simulink model "OR_6s_30l"  (R2023b)
settings: Solver=VariableStepAuto  StartTime=0.0  StopTime=10.0  RelTol=1e-3
libraries: ABB_UPPAAL_Library x76
(part 1 of 2)
settings Model: Creator=francescopellei  LastModifiedBy=francescopellei

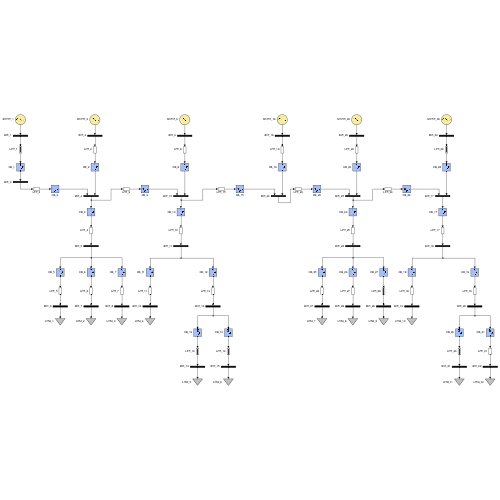
[thumbnail: Simulink's stored preview of the top-level diagram]
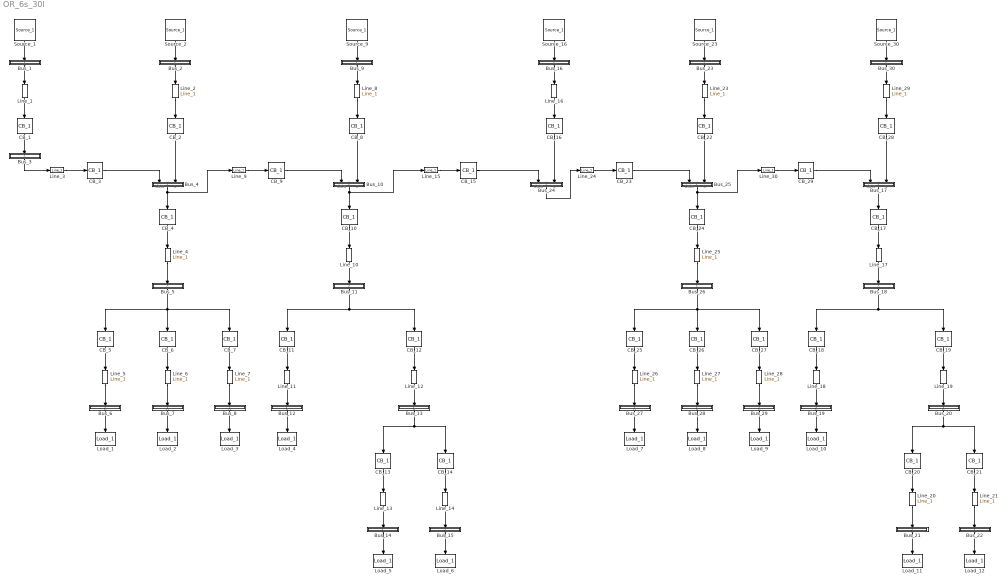
== system OR_6s_30l ==
  Bus_1 : MATLAB Function  TreatAsAtomicUnit=on  mask{MyInitialization=0, Bus_ID=1, Fault_flag=1}
      mask prompts: Bus_ID "Bus ID"; Fault_flag "Fault flag"
      settings: CopyFcn=|
      | Component_Name = get_param(gcb, 'Name');
      | set_param(gcb, 'Bus_ID', num2str(strtrim(extractAfter(Component_Name, '_'))));
      | 
      | blocks = find_system(gcs, 'SearchDepth', 1, 'Type', 'Block');
      | 
      | for k = 1:length(blocks)
      |     if contains(extractAfter(blocks{k,1}, '/'), 'Source')
      |         set_param(blocks{k}, 'BackgroundColor', '[0.929000, 0.490000, 0.439000]');
      |     end
      | end
      settings: NameChangeFcn=|
      | Component_Name = get_param(gcb, 'Name');
      | old_ID = get_param(gcb, 'Bus_ID');
      | 
      | pattern = '_\d+';
      | match = regexp(Component_Name, pattern, 'match');
      | 
      | if ~isempty(match)
      |     if ~isequal(old_ID, num2str(strtrim(extractAfter(Component_Name, '_'))))
      |         set_param(gcb, 'Bus_ID', num2str(strtrim(extractAfter(Component_Name, '_'))));
      |     end
      | else
      |     newName = [Component_Name '_' old_ID];
      |     set_param(gcb, 'Name', newName);
      | end
      | 
      | if ~isequal(old_ID, get_param(gcb, 'Bus_ID'))
      | 
      |     data = get_param(gcb, 'PortConnectivity');
      |     for i = 1:numel(data)
      |         sourceHandle = data(i,1).SrcBlock;
      |         if ~isempty(sourceHandle) && sourceHandle ~= -1
      |             sourceParams = get_param(sourceHandle, 'DialogParameters');
      |             fn = fieldnames(sourceParams);
      |             if contains(fn{2}, 'Source')
      |                 Bus_ID = get_param(gcb, 'Bus_ID');
      |                 set_param(sourceHandle, 'Source_ID', Bus_ID);
      |             end
      |         end
      |     end
      | 
      |     blocks = find_system(gcs, 'SearchDepth', 1, 'Type', 'Block');
      | 
      |     for k = 1:length(blocks)
      |         if contains(extractAfter(blocks{k,1}, '/'), 'Source')
      |             set_param(blocks{k}, 'BackgroundColor', '[0.929000, 0.490000, 0.439000]');
      |         end
      |     end
      | 
      | end
      settings: PreDeleteFcn=|
      | blocks = find_system(gcs, 'SearchDepth', 1, 'Type', 'Block');
      | 
      | for k = 1:length(blocks)
      |     if contains(extractAfter(blocks{k,1}, '/'), 'Source')
      |         set_param(blocks{k}, 'BackgroundColor', '[0.929000, 0.490000, 0.439000]');
      |     end
      | end
  Bus_10 : MATLAB Function  TreatAsAtomicUnit=on  mask{MyInitialization=0, Bus_ID=10, Fault_flag=1}
      mask prompts: Bus_ID "Bus ID"; Fault_flag "Fault flag"
      settings: CopyFcn=|
      | Component_Name = get_param(gcb, 'Name');
      | set_param(gcb, 'Bus_ID', num2str(strtrim(extractAfter(Component_Name, '_'))));
      | 
      | blocks = find_system(gcs, 'SearchDepth', 1, 'Type', 'Block');
      | 
      | for k = 1:length(blocks)
      |     if contains(extractAfter(blocks{k,1}, '/'), 'Source')
      |         set_param(blocks{k}, 'BackgroundColor', '[0.929000, 0.490000, 0.439000]');
      |     end
      | end
      settings: NameChangeFcn=|
      | Component_Name = get_param(gcb, 'Name');
      | old_ID = get_param(gcb, 'Bus_ID');
      | 
      | pattern = '_\d+';
      | match = regexp(Component_Name, pattern, 'match');
      | 
      | if ~isempty(match)
      |     if ~isequal(old_ID, num2str(strtrim(extractAfter(Component_Name, '_'))))
      |         set_param(gcb, 'Bus_ID', num2str(strtrim(extractAfter(Component_Name, '_'))));
      |     end
      | else
      |     newName = [Component_Name '_' old_ID];
      |     set_param(gcb, 'Name', newName);
      | end
      | 
      | if ~isequal(old_ID, get_param(gcb, 'Bus_ID'))
      | 
      |     data = get_param(gcb, 'PortConnectivity');
      |     for i = 1:numel(data)
      |         sourceHandle = data(i,1).SrcBlock;
      |         if ~isempty(sourceHandle) && sourceHandle ~= -1
      |             sourceParams = get_param(sourceHandle, 'DialogParameters');
      |             fn = fieldnames(sourceParams);
      |             if contains(fn{2}, 'Source')
      |                 Bus_ID = get_param(gcb, 'Bus_ID');
      |                 set_param(sourceHandle, 'Source_ID', Bus_ID);
      |             end
      |         end
      |     end
      | 
      |     blocks = find_system(gcs, 'SearchDepth', 1, 'Type', 'Block');
      | 
      |     for k = 1:length(blocks)
      |         if contains(extractAfter(blocks{k,1}, '/'), 'Source')
      |             set_param(blocks{k}, 'BackgroundColor', '[0.929000, 0.490000, 0.439000]');
      |         end
      |     end
      | 
      | end
      settings: PreDeleteFcn=|
      | blocks = find_system(gcs, 'SearchDepth', 1, 'Type', 'Block');
      | 
      | for k = 1:length(blocks)
      |     if contains(extractAfter(blocks{k,1}, '/'), 'Source')
      |         set_param(blocks{k}, 'BackgroundColor', '[0.929000, 0.490000, 0.439000]');
      |     end
      | end
  Bus_11 : MATLAB Function  TreatAsAtomicUnit=on  mask{MyInitialization=0, Bus_ID=11, Fault_flag=1}
      mask prompts: Bus_ID "Bus ID"; Fault_flag "Fault flag"
      settings: CopyFcn=|
      | Component_Name = get_param(gcb, 'Name');
      | set_param(gcb, 'Bus_ID', num2str(strtrim(extractAfter(Component_Name, '_'))));
      | 
      | blocks = find_system(gcs, 'SearchDepth', 1, 'Type', 'Block');
      | 
      | for k = 1:length(blocks)
      |     if contains(extractAfter(blocks{k,1}, '/'), 'Source')
      |         set_param(blocks{k}, 'BackgroundColor', '[0.929000, 0.490000, 0.439000]');
      |     end
      | end
      settings: NameChangeFcn=|
      | Component_Name = get_param(gcb, 'Name');
      | old_ID = get_param(gcb, 'Bus_ID');
      | 
      | pattern = '_\d+';
      | match = regexp(Component_Name, pattern, 'match');
      | 
      | if ~isempty(match)
      |     if ~isequal(old_ID, num2str(strtrim(extractAfter(Component_Name, '_'))))
      |         set_param(gcb, 'Bus_ID', num2str(strtrim(extractAfter(Component_Name, '_'))));
      |     end
      | else
      |     newName = [Component_Name '_' old_ID];
      |     set_param(gcb, 'Name', newName);
      | end
      | 
      | if ~isequal(old_ID, get_param(gcb, 'Bus_ID'))
      | 
      |     data = get_param(gcb, 'PortConnectivity');
      |     for i = 1:numel(data)
      |         sourceHandle = data(i,1).SrcBlock;
      |         if ~isempty(sourceHandle) && sourceHandle ~= -1
      |             sourceParams = get_param(sourceHandle, 'DialogParameters');
      |             fn = fieldnames(sourceParams);
      |             if contains(fn{2}, 'Source')
      |                 Bus_ID = get_param(gcb, 'Bus_ID');
      |                 set_param(sourceHandle, 'Source_ID', Bus_ID);
      |             end
      |         end
      |     end
      | 
      |     blocks = find_system(gcs, 'SearchDepth', 1, 'Type', 'Block');
      | 
      |     for k = 1:length(blocks)
      |         if contains(extractAfter(blocks{k,1}, '/'), 'Source')
      |             set_param(blocks{k}, 'BackgroundColor', '[0.929000, 0.490000, 0.439000]');
      |         end
      |     end
      | 
      | end
      settings: PreDeleteFcn=|
      | blocks = find_system(gcs, 'SearchDepth', 1, 'Type', 'Block');
      | 
      | for k = 1:length(blocks)
      |     if contains(extractAfter(blocks{k,1}, '/'), 'Source')
      |         set_param(blocks{k}, 'BackgroundColor', '[0.929000, 0.490000, 0.439000]');
      |     end
      | end
  Bus_12 : MATLAB Function  TreatAsAtomicUnit=on  mask{MyInitialization=0, Bus_ID=12, Fault_flag=1}
      mask prompts: Bus_ID "Bus ID"; Fault_flag "Fault flag"
      settings: CopyFcn=|
      | Component_Name = get_param(gcb, 'Name');
      | set_param(gcb, 'Bus_ID', num2str(strtrim(extractAfter(Component_Name, '_'))));
      | 
      | blocks = find_system(gcs, 'SearchDepth', 1, 'Type', 'Block');
      | 
      | for k = 1:length(blocks)
      |     if contains(extractAfter(blocks{k,1}, '/'), 'Source')
      |         set_param(blocks{k}, 'BackgroundColor', '[0.929000, 0.490000, 0.439000]');
      |     end
      | end
      settings: NameChangeFcn=|
      | Component_Name = get_param(gcb, 'Name');
      | old_ID = get_param(gcb, 'Bus_ID');
      | 
      | pattern = '_\d+';
      | match = regexp(Component_Name, pattern, 'match');
      | 
      | if ~isempty(match)
      |     if ~isequal(old_ID, num2str(strtrim(extractAfter(Component_Name, '_'))))
      |         set_param(gcb, 'Bus_ID', num2str(strtrim(extractAfter(Component_Name, '_'))));
      |     end
      | else
      |     newName = [Component_Name '_' old_ID];
      |     set_param(gcb, 'Name', newName);
      | end
      | 
      | if ~isequal(old_ID, get_param(gcb, 'Bus_ID'))
      | 
      |     data = get_param(gcb, 'PortConnectivity');
      |     for i = 1:numel(data)
      |         sourceHandle = data(i,1).SrcBlock;
      |         if ~isempty(sourceHandle) && sourceHandle ~= -1
      |             sourceParams = get_param(sourceHandle, 'DialogParameters');
      |             fn = fieldnames(sourceParams);
      |             if contains(fn{2}, 'Source')
      |                 Bus_ID = get_param(gcb, 'Bus_ID');
      |                 set_param(sourceHandle, 'Source_ID', Bus_ID);
      |             end
      |         end
      |     end
      | 
      |     blocks = find_system(gcs, 'SearchDepth', 1, 'Type', 'Block');
      | 
      |     for k = 1:length(blocks)
      |         if contains(extractAfter(blocks{k,1}, '/'), 'Source')
      |             set_param(blocks{k}, 'BackgroundColor', '[0.929000, 0.490000, 0.439000]');
      |         end
      |     end
      | 
      | end
      settings: PreDeleteFcn=|
      | blocks = find_system(gcs, 'SearchDepth', 1, 'Type', 'Block');
      | 
      | for k = 1:length(blocks)
      |     if contains(extractAfter(blocks{k,1}, '/'), 'Source')
      |         set_param(blocks{k}, 'BackgroundColor', '[0.929000, 0.490000, 0.439000]');
      |     end
      | end
  Bus_13 : MATLAB Function  TreatAsAtomicUnit=on  mask{MyInitialization=0, Bus_ID=13, Fault_flag=1}
      mask prompts: Bus_ID "Bus ID"; Fault_flag "Fault flag"
      settings: CopyFcn=|
      | Component_Name = get_param(gcb, 'Name');
      | set_param(gcb, 'Bus_ID', num2str(strtrim(extractAfter(Component_Name, '_'))));
      | 
      | blocks = find_system(gcs, 'SearchDepth', 1, 'Type', 'Block');
      | 
      | for k = 1:length(blocks)
      |     if contains(extractAfter(blocks{k,1}, '/'), 'Source')
      |         set_param(blocks{k}, 'BackgroundColor', '[0.929000, 0.490000, 0.439000]');
      |     end
      | end
      settings: NameChangeFcn=|
      | Component_Name = get_param(gcb, 'Name');
      | old_ID = get_param(gcb, 'Bus_ID');
      | 
      | pattern = '_\d+';
      | match = regexp(Component_Name, pattern, 'match');
      | 
      | if ~isempty(match)
      |     if ~isequal(old_ID, num2str(strtrim(extractAfter(Component_Name, '_'))))
      |         set_param(gcb, 'Bus_ID', num2str(strtrim(extractAfter(Component_Name, '_'))));
      |     end
      | else
      |     newName = [Component_Name '_' old_ID];
      |     set_param(gcb, 'Name', newName);
      | end
      | 
      | if ~isequal(old_ID, get_param(gcb, 'Bus_ID'))
      | 
      |     data = get_param(gcb, 'PortConnectivity');
      |     for i = 1:numel(data)
      |         sourceHandle = data(i,1).SrcBlock;
      |         if ~isempty(sourceHandle) && sourceHandle ~= -1
      |             sourceParams = get_param(sourceHandle, 'DialogParameters');
      |             fn = fieldnames(sourceParams);
      |             if contains(fn{2}, 'Source')
      |                 Bus_ID = get_param(gcb, 'Bus_ID');
      |                 set_param(sourceHandle, 'Source_ID', Bus_ID);
      |             end
      |         end
      |     end
      | 
      |     blocks = find_system(gcs, 'SearchDepth', 1, 'Type', 'Block');
      | 
      |     for k = 1:length(blocks)
      |         if contains(extractAfter(blocks{k,1}, '/'), 'Source')
      |             set_param(blocks{k}, 'BackgroundColor', '[0.929000, 0.490000, 0.439000]');
      |         end
      |     end
      | 
      | end
      settings: PreDeleteFcn=|
      | blocks = find_system(gcs, 'SearchDepth', 1, 'Type', 'Block');
      | 
      | for k = 1:length(blocks)
      |     if contains(extractAfter(blocks{k,1}, '/'), 'Source')
      |         set_param(blocks{k}, 'BackgroundColor', '[0.929000, 0.490000, 0.439000]');
      |     end
      | end
  Bus_14 : MATLAB Function  TreatAsAtomicUnit=on  mask{MyInitialization=0, Bus_ID=14, Fault_flag=1}
      mask prompts: Bus_ID "Bus ID"; Fault_flag "Fault flag"
      settings: CopyFcn=|
      | Component_Name = get_param(gcb, 'Name');
      | set_param(gcb, 'Bus_ID', num2str(strtrim(extractAfter(Component_Name, '_'))));
      | 
      | blocks = find_system(gcs, 'SearchDepth', 1, 'Type', 'Block');
      | 
      | for k = 1:length(blocks)
      |     if contains(extractAfter(blocks{k,1}, '/'), 'Source')
      |         set_param(blocks{k}, 'BackgroundColor', '[0.929000, 0.490000, 0.439000]');
      |     end
      | end
      settings: NameChangeFcn=|
      | Component_Name = get_param(gcb, 'Name');
      | old_ID = get_param(gcb, 'Bus_ID');
      | 
      | pattern = '_\d+';
      | match = regexp(Component_Name, pattern, 'match');
      | 
      | if ~isempty(match)
      |     if ~isequal(old_ID, num2str(strtrim(extractAfter(Component_Name, '_'))))
      |         set_param(gcb, 'Bus_ID', num2str(strtrim(extractAfter(Component_Name, '_'))));
      |     end
      | else
      |     newName = [Component_Name '_' old_ID];
      |     set_param(gcb, 'Name', newName);
      | end
      | 
      | if ~isequal(old_ID, get_param(gcb, 'Bus_ID'))
      | 
      |     data = get_param(gcb, 'PortConnectivity');
      |     for i = 1:numel(data)
      |         sourceHandle = data(i,1).SrcBlock;
      |         if ~isempty(sourceHandle) && sourceHandle ~= -1
      |             sourceParams = get_param(sourceHandle, 'DialogParameters');
      |             fn = fieldnames(sourceParams);
      |             if contains(fn{2}, 'Source')
      |                 Bus_ID = get_param(gcb, 'Bus_ID');
      |                 set_param(sourceHandle, 'Source_ID', Bus_ID);
      |             end
      |         end
      |     end
      | 
      |     blocks = find_system(gcs, 'SearchDepth', 1, 'Type', 'Block');
      | 
      |     for k = 1:length(blocks)
      |         if contains(extractAfter(blocks{k,1}, '/'), 'Source')
      |             set_param(blocks{k}, 'BackgroundColor', '[0.929000, 0.490000, 0.439000]');
      |         end
      |     end
      | 
      | end
      settings: PreDeleteFcn=|
      | blocks = find_system(gcs, 'SearchDepth', 1, 'Type', 'Block');
      | 
      | for k = 1:length(blocks)
      |     if contains(extractAfter(blocks{k,1}, '/'), 'Source')
      |         set_param(blocks{k}, 'BackgroundColor', '[0.929000, 0.490000, 0.439000]');
      |     end
      | end
  Bus_15 : MATLAB Function  TreatAsAtomicUnit=on  mask{MyInitialization=0, Bus_ID=15, Fault_flag=1}
      mask prompts: Bus_ID "Bus ID"; Fault_flag "Fault flag"
      settings: CopyFcn=|
      | Component_Name = get_param(gcb, 'Name');
      | set_param(gcb, 'Bus_ID', num2str(strtrim(extractAfter(Component_Name, '_'))));
      | 
      | blocks = find_system(gcs, 'SearchDepth', 1, 'Type', 'Block');
      | 
      | for k = 1:length(blocks)
      |     if contains(extractAfter(blocks{k,1}, '/'), 'Source')
      |         set_param(blocks{k}, 'BackgroundColor', '[0.929000, 0.490000, 0.439000]');
      |     end
      | end
      settings: NameChangeFcn=|
      | Component_Name = get_param(gcb, 'Name');
      | old_ID = get_param(gcb, 'Bus_ID');
      | 
      | pattern = '_\d+';
      | match = regexp(Component_Name, pattern, 'match');
      | 
      | if ~isempty(match)
      |     if ~isequal(old_ID, num2str(strtrim(extractAfter(Component_Name, '_'))))
      |         set_param(gcb, 'Bus_ID', num2str(strtrim(extractAfter(Component_Name, '_'))));
      |     end
      | else
      |     newName = [Component_Name '_' old_ID];
      |     set_param(gcb, 'Name', newName);
      | end
      | 
      | if ~isequal(old_ID, get_param(gcb, 'Bus_ID'))
      | 
      |     data = get_param(gcb, 'PortConnectivity');
      |     for i = 1:numel(data)
      |         sourceHandle = data(i,1).SrcBlock;
      |         if ~isempty(sourceHandle) && sourceHandle ~= -1
      |             sourceParams = get_param(sourceHandle, 'DialogParameters');
      |             fn = fieldnames(sourceParams);
      |             if contains(fn{2}, 'Source')
      |                 Bus_ID = get_param(gcb, 'Bus_ID');
      |                 set_param(sourceHandle, 'Source_ID', Bus_ID);
      |             end
      |         end
      |     end
      | 
      |     blocks = find_system(gcs, 'SearchDepth', 1, 'Type', 'Block');
      | 
      |     for k = 1:length(blocks)
      |         if contains(extractAfter(blocks{k,1}, '/'), 'Source')
      |             set_param(blocks{k}, 'BackgroundColor', '[0.929000, 0.490000, 0.439000]');
      |         end
      |     end
      | 
      | end
      settings: PreDeleteFcn=|
      | blocks = find_system(gcs, 'SearchDepth', 1, 'Type', 'Block');
      | 
      | for k = 1:length(blocks)
      |     if contains(extractAfter(blocks{k,1}, '/'), 'Source')
      |         set_param(blocks{k}, 'BackgroundColor', '[0.929000, 0.490000, 0.439000]');
      |     end
      | end
  Bus_16 : MATLAB Function  TreatAsAtomicUnit=on  mask{MyInitialization=0, Bus_ID=16, Fault_flag=1}
      mask prompts: Bus_ID "Bus ID"; Fault_flag "Fault flag"
      settings: CopyFcn=|
      | Component_Name = get_param(gcb, 'Name');
      | set_param(gcb, 'Bus_ID', num2str(strtrim(extractAfter(Component_Name, '_'))));
      | 
      | blocks = find_system(gcs, 'SearchDepth', 1, 'Type', 'Block');
      | 
      | for k = 1:length(blocks)
      |     if contains(extractAfter(blocks{k,1}, '/'), 'Source')
      |         set_param(blocks{k}, 'BackgroundColor', '[0.929000, 0.490000, 0.439000]');
      |     end
      | end
      settings: NameChangeFcn=|
      | Component_Name = get_param(gcb, 'Name');
      | old_ID = get_param(gcb, 'Bus_ID');
      | 
      | pattern = '_\d+';
      | match = regexp(Component_Name, pattern, 'match');
      | 
      | if ~isempty(match)
      |     if ~isequal(old_ID, num2str(strtrim(extractAfter(Component_Name, '_'))))
      |         set_param(gcb, 'Bus_ID', num2str(strtrim(extractAfter(Component_Name, '_'))));
      |     end
      | else
      |     newName = [Component_Name '_' old_ID];
      |     set_param(gcb, 'Name', newName);
      | end
      | 
      | if ~isequal(old_ID, get_param(gcb, 'Bus_ID'))
      | 
      |     data = get_param(gcb, 'PortConnectivity');
      |     for i = 1:numel(data)
      |         sourceHandle = data(i,1).SrcBlock;
      |         if ~isempty(sourceHandle) && sourceHandle ~= -1
      |             sourceParams = get_param(sourceHandle, 'DialogParameters');
      |             fn = fieldnames(sourceParams);
      |             if contains(fn{2}, 'Source')
      |                 Bus_ID = get_param(gcb, 'Bus_ID');
      |                 set_param(sourceHandle, 'Source_ID', Bus_ID);
      |             end
      |         end
      |     end
      | 
      |     blocks = find_system(gcs, 'SearchDepth', 1, 'Type', 'Block');
      | 
      |     for k = 1:length(blocks)
      |         if contains(extractAfter(blocks{k,1}, '/'), 'Source')
      |             set_param(blocks{k}, 'BackgroundColor', '[0.929000, 0.490000, 0.439000]');
      |         end
      |     end
      | 
      | end
      settings: PreDeleteFcn=|
      | blocks = find_system(gcs, 'SearchDepth', 1, 'Type', 'Block');
      | 
      | for k = 1:length(blocks)
      |     if contains(extractAfter(blocks{k,1}, '/'), 'Source')
      |         set_param(blocks{k}, 'BackgroundColor', '[0.929000, 0.490000, 0.439000]');
      |     end
      | end
  Bus_17 : MATLAB Function  TreatAsAtomicUnit=on  mask{MyInitialization=0, Bus_ID=17, Fault_flag=1}
      mask prompts: Bus_ID "Bus ID"; Fault_flag "Fault flag"
      settings: CopyFcn=|
      | Component_Name = get_param(gcb, 'Name');
      | set_param(gcb, 'Bus_ID', num2str(strtrim(extractAfter(Component_Name, '_'))));
      | 
      | blocks = find_system(gcs, 'SearchDepth', 1, 'Type', 'Block');
      | 
      | for k = 1:length(blocks)
      |     if contains(extractAfter(blocks{k,1}, '/'), 'Source')
      |         set_param(blocks{k}, 'BackgroundColor', '[0.929000, 0.490000, 0.439000]');
      |     end
      | end
      settings: NameChangeFcn=|
      | Component_Name = get_param(gcb, 'Name');
      | old_ID = get_param(gcb, 'Bus_ID');
      | 
      | pattern = '_\d+';
      | match = regexp(Component_Name, pattern, 'match');
      | 
      | if ~isempty(match)
      |     if ~isequal(old_ID, num2str(strtrim(extractAfter(Component_Name, '_'))))
      |         set_param(gcb, 'Bus_ID', num2str(strtrim(extractAfter(Component_Name, '_'))));
      |     end
      | else
      |     newName = [Component_Name '_' old_ID];
      |     set_param(gcb, 'Name', newName);
      | end
      | 
      | if ~isequal(old_ID, get_param(gcb, 'Bus_ID'))
      | 
      |     data = get_param(gcb, 'PortConnectivity');
      |     for i = 1:numel(data)
      |         sourceHandle = data(i,1).SrcBlock;
      |         if ~isempty(sourceHandle) && sourceHandle ~= -1
      |             sourceParams = get_param(sourceHandle, 'DialogParameters');
      |             fn = fieldnames(sourceParams);
      |             if contains(fn{2}, 'Source')
      |                 Bus_ID = get_param(gcb, 'Bus_ID');
      |                 set_param(sourceHandle, 'Source_ID', Bus_ID);
      |             end
      |         end
      |     end
      | 
      |     blocks = find_system(gcs, 'SearchDepth', 1, 'Type', 'Block');
      | 
      |     for k = 1:length(blocks)
      |         if contains(extractAfter(blocks{k,1}, '/'), 'Source')
      |             set_param(blocks{k}, 'BackgroundColor', '[0.929000, 0.490000, 0.439000]');
      |         end
      |     end
      | 
      | end
      settings: PreDeleteFcn=|
      | blocks = find_system(gcs, 'SearchDepth', 1, 'Type', 'Block');
      | 
      | for k = 1:length(blocks)
      |     if contains(extractAfter(blocks{k,1}, '/'), 'Source')
      |         set_param(blocks{k}, 'BackgroundColor', '[0.929000, 0.490000, 0.439000]');
      |     end
      | end
  Bus_18 : MATLAB Function  TreatAsAtomicUnit=on  mask{MyInitialization=0, Bus_ID=18, Fault_flag=1}
      mask prompts: Bus_ID "Bus ID"; Fault_flag "Fault flag"
      settings: CopyFcn=|
      | Component_Name = get_param(gcb, 'Name');
      | set_param(gcb, 'Bus_ID', num2str(strtrim(extractAfter(Component_Name, '_'))));
      | 
      | blocks = find_system(gcs, 'SearchDepth', 1, 'Type', 'Block');
      | 
      | for k = 1:length(blocks)
      |     if contains(extractAfter(blocks{k,1}, '/'), 'Source')
      |         set_param(blocks{k}, 'BackgroundColor', '[0.929000, 0.490000, 0.439000]');
      |     end
      | end
      settings: NameChangeFcn=|
      | Component_Name = get_param(gcb, 'Name');
      | old_ID = get_param(gcb, 'Bus_ID');
      | 
      | pattern = '_\d+';
      | match = regexp(Component_Name, pattern, 'match');
      | 
      | if ~isempty(match)
      |     if ~isequal(old_ID, num2str(strtrim(extractAfter(Component_Name, '_'))))
      |         set_param(gcb, 'Bus_ID', num2str(strtrim(extractAfter(Component_Name, '_'))));
      |     end
      | else
      |     newName = [Component_Name '_' old_ID];
      |     set_param(gcb, 'Name', newName);
      | end
      | 
      | if ~isequal(old_ID, get_param(gcb, 'Bus_ID'))
      | 
      |     data = get_param(gcb, 'PortConnectivity');
      |     for i = 1:numel(data)
      |         sourceHandle = data(i,1).SrcBlock;
      |         if ~isempty(sourceHandle) && sourceHandle ~= -1
      |             sourceParams = get_param(sourceHandle, 'DialogParameters');
      |             fn = fieldnames(sourceParams);
      |             if contains(fn{2}, 'Source')
      |                 Bus_ID = get_param(gcb, 'Bus_ID');
      |                 set_param(sourceHandle, 'Source_ID', Bus_ID);
      |             end
      |         end
      |     end
      | 
      |     blocks = find_system(gcs, 'SearchDepth', 1, 'Type', 'Block');
      | 
      |     for k = 1:length(blocks)
      |         if contains(extractAfter(blocks{k,1}, '/'), 'Source')
      |             set_param(blocks{k}, 'BackgroundColor', '[0.929000, 0.490000, 0.439000]');
      |         end
      |     end
      | 
      | end
      settings: PreDeleteFcn=|
      | blocks = find_system(gcs, 'SearchDepth', 1, 'Type', 'Block');
      | 
      | for k = 1:length(blocks)
      |     if contains(extractAfter(blocks{k,1}, '/'), 'Source')
      |         set_param(blocks{k}, 'BackgroundColor', '[0.929000, 0.490000, 0.439000]');
      |     end
      | end
  Bus_19 : MATLAB Function  TreatAsAtomicUnit=on  mask{MyInitialization=0, Bus_ID=19, Fault_flag=1}
      mask prompts: Bus_ID "Bus ID"; Fault_flag "Fault flag"
      settings: CopyFcn=|
      | Component_Name = get_param(gcb, 'Name');
      | set_param(gcb, 'Bus_ID', num2str(strtrim(extractAfter(Component_Name, '_'))));
      | 
      | blocks = find_system(gcs, 'SearchDepth', 1, 'Type', 'Block');
      | 
      | for k = 1:length(blocks)
      |     if contains(extractAfter(blocks{k,1}, '/'), 'Source')
      |         set_param(blocks{k}, 'BackgroundColor', '[0.929000, 0.490000, 0.439000]');
      |     end
      | end
      settings: NameChangeFcn=|
      | Component_Name = get_param(gcb, 'Name');
      | old_ID = get_param(gcb, 'Bus_ID');
      | 
      | pattern = '_\d+';
      | match = regexp(Component_Name, pattern, 'match');
      | 
      | if ~isempty(match)
      |     if ~isequal(old_ID, num2str(strtrim(extractAfter(Component_Name, '_'))))
      |         set_param(gcb, 'Bus_ID', num2str(strtrim(extractAfter(Component_Name, '_'))));
      |     end
      | else
      |     newName = [Component_Name '_' old_ID];
      |     set_param(gcb, 'Name', newName);
      | end
      | 
      | if ~isequal(old_ID, get_param(gcb, 'Bus_ID'))
      | 
      |     data = get_param(gcb, 'PortConnectivity');
      |     for i = 1:numel(data)
      |         sourceHandle = data(i,1).SrcBlock;
      |         if ~isempty(sourceHandle) && sourceHandle ~= -1
      |             sourceParams = get_param(sourceHandle, 'DialogParameters');
      |             fn = fieldnames(sourceParams);
      |             if contains(fn{2}, 'Source')
      |                 Bus_ID = get_param(gcb, 'Bus_ID');
      |                 set_param(sourceHandle, 'Source_ID', Bus_ID);
      |             end
      |         end
      |     end
      | 
      |     blocks = find_system(gcs, 'SearchDepth', 1, 'Type', 'Block');
      | 
      |     for k = 1:length(blocks)
      |         if contains(extractAfter(blocks{k,1}, '/'), 'Source')
      |             set_param(blocks{k}, 'BackgroundColor', '[0.929000, 0.490000, 0.439000]');
      |         end
      |     end
      | 
      | end
      settings: PreDeleteFcn=|
      | blocks = find_system(gcs, 'SearchDepth', 1, 'Type', 'Block');
      | 
      | for k = 1:length(blocks)
      |     if contains(extractAfter(blocks{k,1}, '/'), 'Source')
      |         set_param(blocks{k}, 'BackgroundColor', '[0.929000, 0.490000, 0.439000]');
      |     end
      | end
  Bus_2 : MATLAB Function  TreatAsAtomicUnit=on  mask{MyInitialization=0, Bus_ID=2, Fault_flag=1}
      mask prompts: Bus_ID "Bus ID"; Fault_flag "Fault flag"
      settings: CopyFcn=|
      | Component_Name = get_param(gcb, 'Name');
      | set_param(gcb, 'Bus_ID', num2str(strtrim(extractAfter(Component_Name, '_'))));
      | 
      | blocks = find_system(gcs, 'SearchDepth', 1, 'Type', 'Block');
      | 
      | for k = 1:length(blocks)
      |     if contains(extractAfter(blocks{k,1}, '/'), 'Source')
      |         set_param(blocks{k}, 'BackgroundColor', '[0.929000, 0.490000, 0.439000]');
      |     end
      | end
      settings: NameChangeFcn=|
      | Component_Name = get_param(gcb, 'Name');
      | old_ID = get_param(gcb, 'Bus_ID');
      | 
      | pattern = '_\d+';
      | match = regexp(Component_Name, pattern, 'match');
      | 
      | if ~isempty(match)
      |     if ~isequal(old_ID, num2str(strtrim(extractAfter(Component_Name, '_'))))
      |         set_param(gcb, 'Bus_ID', num2str(strtrim(extractAfter(Component_Name, '_'))));
      |     end
      | else
      |     newName = [Component_Name '_' old_ID];
      |     set_param(gcb, 'Name', newName);
      | end
      | 
      | if ~isequal(old_ID, get_param(gcb, 'Bus_ID'))
      | 
      |     data = get_param(gcb, 'PortConnectivity');
      |     for i = 1:numel(data)
      |         sourceHandle = data(i,1).SrcBlock;
      |         if ~isempty(sourceHandle) && sourceHandle ~= -1
      |             sourceParams = get_param(sourceHandle, 'DialogParameters');
      |             fn = fieldnames(sourceParams);
      |             if contains(fn{2}, 'Source')
      |                 Bus_ID = get_param(gcb, 'Bus_ID');
      |                 set_param(sourceHandle, 'Source_ID', Bus_ID);
      |             end
      |         end
      |     end
      | 
      |     blocks = find_system(gcs, 'SearchDepth', 1, 'Type', 'Block');
      | 
      |     for k = 1:length(blocks)
      |         if contains(extractAfter(blocks{k,1}, '/'), 'Source')
      |             set_param(blocks{k}, 'BackgroundColor', '[0.929000, 0.490000, 0.439000]');
      |         end
      |     end
      | 
      | end
      settings: PreDeleteFcn=|
      | blocks = find_system(gcs, 'SearchDepth', 1, 'Type', 'Block');
      | 
      | for k = 1:length(blocks)
      |     if contains(extractAfter(blocks{k,1}, '/'), 'Source')
      |         set_param(blocks{k}, 'BackgroundColor', '[0.929000, 0.490000, 0.439000]');
      |     end
      | end
  Bus_20 : MATLAB Function  TreatAsAtomicUnit=on  mask{MyInitialization=0, Bus_ID=20, Fault_flag=1}
      mask prompts: Bus_ID "Bus ID"; Fault_flag "Fault flag"
      settings: CopyFcn=|
      | Component_Name = get_param(gcb, 'Name');
      | set_param(gcb, 'Bus_ID', num2str(strtrim(extractAfter(Component_Name, '_'))));
      | 
      | blocks = find_system(gcs, 'SearchDepth', 1, 'Type', 'Block');
      | 
      | for k = 1:length(blocks)
      |     if contains(extractAfter(blocks{k,1}, '/'), 'Source')
      |         set_param(blocks{k}, 'BackgroundColor', '[0.929000, 0.490000, 0.439000]');
      |     end
      | end
      settings: NameChangeFcn=|
      | Component_Name = get_param(gcb, 'Name');
      | old_ID = get_param(gcb, 'Bus_ID');
      | 
      | pattern = '_\d+';
      | match = regexp(Component_Name, pattern, 'match');
      | 
      | if ~isempty(match)
      |     if ~isequal(old_ID, num2str(strtrim(extractAfter(Component_Name, '_'))))
      |         set_param(gcb, 'Bus_ID', num2str(strtrim(extractAfter(Component_Name, '_'))));
      |     end
      | else
      |     newName = [Component_Name '_' old_ID];
      |     set_param(gcb, 'Name', newName);
      | end
      | 
      | if ~isequal(old_ID, get_param(gcb, 'Bus_ID'))
      | 
      |     data = get_param(gcb, 'PortConnectivity');
      |     for i = 1:numel(data)
      |         sourceHandle = data(i,1).SrcBlock;
      |         if ~isempty(sourceHandle) && sourceHandle ~= -1
      |             sourceParams = get_param(sourceHandle, 'DialogParameters');
      |             fn = fieldnames(sourceParams);
      |             if contains(fn{2}, 'Source')
      |                 Bus_ID = get_param(gcb, 'Bus_ID');
      |                 set_param(sourceHandle, 'Source_ID', Bus_ID);
      |             end
      |         end
      |     end
      | 
      |     blocks = find_system(gcs, 'SearchDepth', 1, 'Type', 'Block');
      | 
      |     for k = 1:length(blocks)
      |         if contains(extractAfter(blocks{k,1}, '/'), 'Source')
      |             set_param(blocks{k}, 'BackgroundColor', '[0.929000, 0.490000, 0.439000]');
      |         end
      |     end
      | 
      | end
      settings: PreDeleteFcn=|
      | blocks = find_system(gcs, 'SearchDepth', 1, 'Type', 'Block');
      | 
      | for k = 1:length(blocks)
      |     if contains(extractAfter(blocks{k,1}, '/'), 'Source')
      |         set_param(blocks{k}, 'BackgroundColor', '[0.929000, 0.490000, 0.439000]');
      |     end
      | end
  Bus_21 : MATLAB Function  TreatAsAtomicUnit=on  mask{MyInitialization=0, Bus_ID=21, Fault_flag=1}
      mask prompts: Bus_ID "Bus ID"; Fault_flag "Fault flag"
      settings: CopyFcn=|
      | Component_Name = get_param(gcb, 'Name');
      | set_param(gcb, 'Bus_ID', num2str(strtrim(extractAfter(Component_Name, '_'))));
      | 
      | blocks = find_system(gcs, 'SearchDepth', 1, 'Type', 'Block');
      | 
      | for k = 1:length(blocks)
      |     if contains(extractAfter(blocks{k,1}, '/'), 'Source')
      |         set_param(blocks{k}, 'BackgroundColor', '[0.929000, 0.490000, 0.439000]');
      |     end
      | end
      settings: NameChangeFcn=|
      | Component_Name = get_param(gcb, 'Name');
      | old_ID = get_param(gcb, 'Bus_ID');
      | 
      | pattern = '_\d+';
      | match = regexp(Component_Name, pattern, 'match');
      | 
      | if ~isempty(match)
      |     if ~isequal(old_ID, num2str(strtrim(extractAfter(Component_Name, '_'))))
      |         set_param(gcb, 'Bus_ID', num2str(strtrim(extractAfter(Component_Name, '_'))));
      |     end
      | else
      |     newName = [Component_Name '_' old_ID];
      |     set_param(gcb, 'Name', newName);
      | end
      | 
      | if ~isequal(old_ID, get_param(gcb, 'Bus_ID'))
      | 
      |     data = get_param(gcb, 'PortConnectivity');
      |     for i = 1:numel(data)
      |         sourceHandle = data(i,1).SrcBlock;
      |         if ~isempty(sourceHandle) && sourceHandle ~= -1
      |             sourceParams = get_param(sourceHandle, 'DialogParameters');
      |             fn = fieldnames(sourceParams);
      |             if contains(fn{2}, 'Source')
      |                 Bus_ID = get_param(gcb, 'Bus_ID');
      |                 set_param(sourceHandle, 'Source_ID', Bus_ID);
      |             end
      |         end
      |     end
      | 
      |     blocks = find_system(gcs, 'SearchDepth', 1, 'Type', 'Block');
      | 
      |     for k = 1:length(blocks)
      |         if contains(extractAfter(blocks{k,1}, '/'), 'Source')
      |             set_param(blocks{k}, 'BackgroundColor', '[0.929000, 0.490000, 0.439000]');
      |         end
      |     end
      | 
      | end
      settings: PreDeleteFcn=|
      | blocks = find_system(gcs, 'SearchDepth', 1, 'Type', 'Block');
      | 
      | for k = 1:length(blocks)
      |     if contains(extractAfter(blocks{k,1}, '/'), 'Source')
      |         set_param(blocks{k}, 'BackgroundColor', '[0.929000, 0.490000, 0.439000]');
      |     end
      | end
  Bus_22 : MATLAB Function  TreatAsAtomicUnit=on  mask{MyInitialization=0, Bus_ID=22, Fault_flag=1}
      mask prompts: Bus_ID "Bus ID"; Fault_flag "Fault flag"
      settings: CopyFcn=|
      | Component_Name = get_param(gcb, 'Name');
      | set_param(gcb, 'Bus_ID', num2str(strtrim(extractAfter(Component_Name, '_'))));
      | 
      | blocks = find_system(gcs, 'SearchDepth', 1, 'Type', 'Block');
      | 
      | for k = 1:length(blocks)
      |     if contains(extractAfter(blocks{k,1}, '/'), 'Source')
      |         set_param(blocks{k}, 'BackgroundColor', '[0.929000, 0.490000, 0.439000]');
      |     end
      | end
      settings: NameChangeFcn=|
      | Component_Name = get_param(gcb, 'Name');
      | old_ID = get_param(gcb, 'Bus_ID');
      | 
      | pattern = '_\d+';
      | match = regexp(Component_Name, pattern, 'match');
      | 
      | if ~isempty(match)
      |     if ~isequal(old_ID, num2str(strtrim(extractAfter(Component_Name, '_'))))
      |         set_param(gcb, 'Bus_ID', num2str(strtrim(extractAfter(Component_Name, '_'))));
      |     end
      | else
      |     newName = [Component_Name '_' old_ID];
      |     set_param(gcb, 'Name', newName);
      | end
      | 
      | if ~isequal(old_ID, get_param(gcb, 'Bus_ID'))
      | 
      |     data = get_param(gcb, 'PortConnectivity');
      |     for i = 1:numel(data)
      |         sourceHandle = data(i,1).SrcBlock;
      |         if ~isempty(sourceHandle) && sourceHandle ~= -1
      |             sourceParams = get_param(sourceHandle, 'DialogParameters');
      |             fn = fieldnames(sourceParams);
      |             if contains(fn{2}, 'Source')
      |                 Bus_ID = get_param(gcb, 'Bus_ID');
      |                 set_param(sourceHandle, 'Source_ID', Bus_ID);
      |             end
      |         end
      |     end
      | 
      |     blocks = find_system(gcs, 'SearchDepth', 1, 'Type', 'Block');
      | 
      |     for k = 1:length(blocks)
      |         if contains(extractAfter(blocks{k,1}, '/'), 'Source')
      |             set_param(blocks{k}, 'BackgroundColor', '[0.929000, 0.490000, 0.439000]');
      |         end
      |     end
      | 
      | end
      settings: PreDeleteFcn=|
      | blocks = find_system(gcs, 'SearchDepth', 1, 'Type', 'Block');
      | 
      | for k = 1:length(blocks)
      |     if contains(extractAfter(blocks{k,1}, '/'), 'Source')
      |         set_param(blocks{k}, 'BackgroundColor', '[0.929000, 0.490000, 0.439000]');
      |     end
      | end
  Bus_23 : MATLAB Function  TreatAsAtomicUnit=on  mask{MyInitialization=0, Bus_ID=23, Fault_flag=1}
      mask prompts: Bus_ID "Bus ID"; Fault_flag "Fault flag"
      settings: CopyFcn=|
      | Component_Name = get_param(gcb, 'Name');
      | set_param(gcb, 'Bus_ID', num2str(strtrim(extractAfter(Component_Name, '_'))));
      | 
      | blocks = find_system(gcs, 'SearchDepth', 1, 'Type', 'Block');
      | 
      | for k = 1:length(blocks)
      |     if contains(extractAfter(blocks{k,1}, '/'), 'Source')
      |         set_param(blocks{k}, 'BackgroundColor', '[0.929000, 0.490000, 0.439000]');
      |     end
      | end
      settings: NameChangeFcn=|
      | Component_Name = get_param(gcb, 'Name');
      | old_ID = get_param(gcb, 'Bus_ID');
      | 
      | pattern = '_\d+';
      | match = regexp(Component_Name, pattern, 'match');
      | 
      | if ~isempty(match)
      |     if ~isequal(old_ID, num2str(strtrim(extractAfter(Component_Name, '_'))))
      |         set_param(gcb, 'Bus_ID', num2str(strtrim(extractAfter(Component_Name, '_'))));
      |     end
      | else
      |     newName = [Component_Name '_' old_ID];
      |     set_param(gcb, 'Name', newName);
      | end
      | 
      | if ~isequal(old_ID, get_param(gcb, 'Bus_ID'))
      | 
      |     data = get_param(gcb, 'PortConnectivity');
      |     for i = 1:numel(data)
      |         sourceHandle = data(i,1).SrcBlock;
      |         if ~isempty(sourceHandle) && sourceHandle ~= -1
      |             sourceParams = get_param(sourceHandle, 'DialogParameters');
      |             fn = fieldnames(sourceParams);
      |             if contains(fn{2}, 'Source')
      |                 Bus_ID = get_param(gcb, 'Bus_ID');
      |                 set_param(sourceHandle, 'Source_ID', Bus_ID);
      |             end
      |         end
      |     end
      | 
      |     blocks = find_system(gcs, 'SearchDepth', 1, 'Type', 'Block');
      | 
      |     for k = 1:length(blocks)
      |         if contains(extractAfter(blocks{k,1}, '/'), 'Source')
      |             set_param(blocks{k}, 'BackgroundColor', '[0.929000, 0.490000, 0.439000]');
      |         end
      |     end
      | 
      | end
      settings: PreDeleteFcn=|
      | blocks = find_system(gcs, 'SearchDepth', 1, 'Type', 'Block');
      | 
      | for k = 1:length(blocks)
      |     if contains(extractAfter(blocks{k,1}, '/'), 'Source')
      |         set_param(blocks{k}, 'BackgroundColor', '[0.929000, 0.490000, 0.439000]');
      |     end
      | end
  Bus_24 : MATLAB Function  TreatAsAtomicUnit=on  mask{MyInitialization=0, Bus_ID=24, Fault_flag=1}
      mask prompts: Bus_ID "Bus ID"; Fault_flag "Fault flag"
      settings: CopyFcn=|
      | Component_Name = get_param(gcb, 'Name');
      | set_param(gcb, 'Bus_ID', num2str(strtrim(extractAfter(Component_Name, '_'))));
      | 
      | blocks = find_system(gcs, 'SearchDepth', 1, 'Type', 'Block');
      | 
      | for k = 1:length(blocks)
      |     if contains(extractAfter(blocks{k,1}, '/'), 'Source')
      |         set_param(blocks{k}, 'BackgroundColor', '[0.929000, 0.490000, 0.439000]');
      |     end
      | end
      settings: NameChangeFcn=|
      | Component_Name = get_param(gcb, 'Name');
      | old_ID = get_param(gcb, 'Bus_ID');
      | 
      | pattern = '_\d+';
      | match = regexp(Component_Name, pattern, 'match');
      | 
      | if ~isempty(match)
      |     if ~isequal(old_ID, num2str(strtrim(extractAfter(Component_Name, '_'))))
      |         set_param(gcb, 'Bus_ID', num2str(strtrim(extractAfter(Component_Name, '_'))));
      |     end
      | else
      |     newName = [Component_Name '_' old_ID];
      |     set_param(gcb, 'Name', newName);
      | end
      | 
      | if ~isequal(old_ID, get_param(gcb, 'Bus_ID'))
      | 
      |     data = get_param(gcb, 'PortConnectivity');
      |     for i = 1:numel(data)
      |         sourceHandle = data(i,1).SrcBlock;
      |         if ~isempty(sourceHandle) && sourceHandle ~= -1
      |             sourceParams = get_param(sourceHandle, 'DialogParameters');
      |             fn = fieldnames(sourceParams);
      |             if contains(fn{2}, 'Source')
      |                 Bus_ID = get_param(gcb, 'Bus_ID');
      |                 set_param(sourceHandle, 'Source_ID', Bus_ID);
      |             end
      |         end
      |     end
      | 
      |     blocks = find_system(gcs, 'SearchDepth', 1, 'Type', 'Block');
      | 
      |     for k = 1:length(blocks)
      |         if contains(extractAfter(blocks{k,1}, '/'), 'Source')
      |             set_param(blocks{k}, 'BackgroundColor', '[0.929000, 0.490000, 0.439000]');
      |         end
      |     end
      | 
      | end
      settings: PreDeleteFcn=|
      | blocks = find_system(gcs, 'SearchDepth', 1, 'Type', 'Block');
      | 
      | for k = 1:length(blocks)
      |     if contains(extractAfter(blocks{k,1}, '/'), 'Source')
      |         set_param(blocks{k}, 'BackgroundColor', '[0.929000, 0.490000, 0.439000]');
      |     end
      | end
  Bus_25 : MATLAB Function  TreatAsAtomicUnit=on  mask{MyInitialization=0, Bus_ID=25, Fault_flag=1}
      mask prompts: Bus_ID "Bus ID"; Fault_flag "Fault flag"
      settings: CopyFcn=|
      | Component_Name = get_param(gcb, 'Name');
      | set_param(gcb, 'Bus_ID', num2str(strtrim(extractAfter(Component_Name, '_'))));
      | 
      | blocks = find_system(gcs, 'SearchDepth', 1, 'Type', 'Block');
      | 
      | for k = 1:length(blocks)
      |     if contains(extractAfter(blocks{k,1}, '/'), 'Source')
      |         set_param(blocks{k}, 'BackgroundColor', '[0.929000, 0.490000, 0.439000]');
      |     end
      | end
      settings: NameChangeFcn=|
      | Component_Name = get_param(gcb, 'Name');
      | old_ID = get_param(gcb, 'Bus_ID');
      | 
      | pattern = '_\d+';
      | match = regexp(Component_Name, pattern, 'match');
      | 
      | if ~isempty(match)
      |     if ~isequal(old_ID, num2str(strtrim(extractAfter(Component_Name, '_'))))
      |         set_param(gcb, 'Bus_ID', num2str(strtrim(extractAfter(Component_Name, '_'))));
      |     end
      | else
      |     newName = [Component_Name '_' old_ID];
      |     set_param(gcb, 'Name', newName);
      | end
      | 
      | if ~isequal(old_ID, get_param(gcb, 'Bus_ID'))
      | 
      |     data = get_param(gcb, 'PortConnectivity');
      |     for i = 1:numel(data)
      |         sourceHandle = data(i,1).SrcBlock;
      |         if ~isempty(sourceHandle) && sourceHandle ~= -1
      |             sourceParams = get_param(sourceHandle, 'DialogParameters');
      |             fn = fieldnames(sourceParams);
      |             if contains(fn{2}, 'Source')
      |                 Bus_ID = get_param(gcb, 'Bus_ID');
      |                 set_param(sourceHandle, 'Source_ID', Bus_ID);
      |             end
      |         end
      |     end
      | 
      |     blocks = find_system(gcs, 'SearchDepth', 1, 'Type', 'Block');
      | 
      |     for k = 1:length(blocks)
      |         if contains(extractAfter(blocks{k,1}, '/'), 'Source')
      |             set_param(blocks{k}, 'BackgroundColor', '[0.929000, 0.490000, 0.439000]');
      |         end
      |     end
      | 
      | end
      settings: PreDeleteFcn=|
      | blocks = find_system(gcs, 'SearchDepth', 1, 'Type', 'Block');
      | 
      | for k = 1:length(blocks)
      |     if contains(extractAfter(blocks{k,1}, '/'), 'Source')
      |         set_param(blocks{k}, 'BackgroundColor', '[0.929000, 0.490000, 0.439000]');
      |     end
      | end
  Bus_26 : MATLAB Function  TreatAsAtomicUnit=on  mask{MyInitialization=0, Bus_ID=26, Fault_flag=1}
      mask prompts: Bus_ID "Bus ID"; Fault_flag "Fault flag"
      settings: CopyFcn=|
      | Component_Name = get_param(gcb, 'Name');
      | set_param(gcb, 'Bus_ID', num2str(strtrim(extractAfter(Component_Name, '_'))));
      | 
      | blocks = find_system(gcs, 'SearchDepth', 1, 'Type', 'Block');
      | 
      | for k = 1:length(blocks)
      |     if contains(extractAfter(blocks{k,1}, '/'), 'Source')
      |         set_param(blocks{k}, 'BackgroundColor', '[0.929000, 0.490000, 0.439000]');
      |     end
      | end
      settings: NameChangeFcn=|
      | Component_Name = get_param(gcb, 'Name');
      | old_ID = get_param(gcb, 'Bus_ID');
      | 
      | pattern = '_\d+';
      | match = regexp(Component_Name, pattern, 'match');
      | 
      | if ~isempty(match)
      |     if ~isequal(old_ID, num2str(strtrim(extractAfter(Component_Name, '_'))))
      |         set_param(gcb, 'Bus_ID', num2str(strtrim(extractAfter(Component_Name, '_'))));
      |     end
      | else
      |     newName = [Component_Name '_' old_ID];
      |     set_param(gcb, 'Name', newName);
      | end
      | 
      | if ~isequal(old_ID, get_param(gcb, 'Bus_ID'))
      | 
      |     data = get_param(gcb, 'PortConnectivity');
      |     for i = 1:numel(data)
      |         sourceHandle = data(i,1).SrcBlock;
      |         if ~isempty(sourceHandle) && sourceHandle ~= -1
      |             sourceParams = get_param(sourceHandle, 'DialogParameters');
      |             fn = fieldnames(sourceParams);
      |             if contains(fn{2}, 'Source')
      |                 Bus_ID = get_param(gcb, 'Bus_ID');
      |                 set_param(sourceHandle, 'Source_ID', Bus_ID);
      |             end
      |         end
      |     end
      | 
      |     blocks = find_system(gcs, 'SearchDepth', 1, 'Type', 'Block');
      | 
      |     for k = 1:length(blocks)
      |         if contains(extractAfter(blocks{k,1}, '/'), 'Source')
      |             set_param(blocks{k}, 'BackgroundColor', '[0.929000, 0.490000, 0.439000]');
      |         end
      |     end
      | 
      | end
      settings: PreDeleteFcn=|
      | blocks = find_system(gcs, 'SearchDepth', 1, 'Type', 'Block');
      | 
      | for k = 1:length(blocks)
      |     if contains(extractAfter(blocks{k,1}, '/'), 'Source')
      |         set_param(blocks{k}, 'BackgroundColor', '[0.929000, 0.490000, 0.439000]');
      |     end
      | end
  Bus_27 : MATLAB Function  TreatAsAtomicUnit=on  mask{MyInitialization=0, Bus_ID=27, Fault_flag=1}
      mask prompts: Bus_ID "Bus ID"; Fault_flag "Fault flag"
      settings: CopyFcn=|
      | Component_Name = get_param(gcb, 'Name');
      | set_param(gcb, 'Bus_ID', num2str(strtrim(extractAfter(Component_Name, '_'))));
      | 
      | blocks = find_system(gcs, 'SearchDepth', 1, 'Type', 'Block');
      | 
      | for k = 1:length(blocks)
      |     if contains(extractAfter(blocks{k,1}, '/'), 'Source')
      |         set_param(blocks{k}, 'BackgroundColor', '[0.929000, 0.490000, 0.439000]');
      |     end
      | end
      settings: NameChangeFcn=|
      | Component_Name = get_param(gcb, 'Name');
      | old_ID = get_param(gcb, 'Bus_ID');
      | 
      | pattern = '_\d+';
      | match = regexp(Component_Name, pattern, 'match');
      | 
      | if ~isempty(match)
      |     if ~isequal(old_ID, num2str(strtrim(extractAfter(Component_Name, '_'))))
      |         set_param(gcb, 'Bus_ID', num2str(strtrim(extractAfter(Component_Name, '_'))));
      |     end
      | else
      |     newName = [Component_Name '_' old_ID];
      |     set_param(gcb, 'Name', newName);
      | end
      | 
      | if ~isequal(old_ID, get_param(gcb, 'Bus_ID'))
      | 
      |     data = get_param(gcb, 'PortConnectivity');
      |     for i = 1:numel(data)
      |         sourceHandle = data(i,1).SrcBlock;
      |         if ~isempty(sourceHandle) && sourceHandle ~= -1
      |             sourceParams = get_param(sourceHandle, 'DialogParameters');
      |             fn = fieldnames(sourceParams);
      |             if contains(fn{2}, 'Source')
      |                 Bus_ID = get_param(gcb, 'Bus_ID');
      |                 set_param(sourceHandle, 'Source_ID', Bus_ID);
      |             end
      |         end
      |     end
      | 
      |     blocks = find_system(gcs, 'SearchDepth', 1, 'Type', 'Block');
      | 
      |     for k = 1:length(blocks)
      |         if contains(extractAfter(blocks{k,1}, '/'), 'Source')
      |             set_param(blocks{k}, 'BackgroundColor', '[0.929000, 0.490000, 0.439000]');
      |         end
      |     end
      | 
      | end
      settings: PreDeleteFcn=|
      | blocks = find_system(gcs, 'SearchDepth', 1, 'Type', 'Block');
      | 
      | for k = 1:length(blocks)
      |     if contains(extractAfter(blocks{k,1}, '/'), 'Source')
      |         set_param(blocks{k}, 'BackgroundColor', '[0.929000, 0.490000, 0.439000]');
      |     end
      | end
  Bus_28 : MATLAB Function  TreatAsAtomicUnit=on  mask{MyInitialization=0, Bus_ID=28, Fault_flag=1}
      mask prompts: Bus_ID "Bus ID"; Fault_flag "Fault flag"
      settings: CopyFcn=|
      | Component_Name = get_param(gcb, 'Name');
      | set_param(gcb, 'Bus_ID', num2str(strtrim(extractAfter(Component_Name, '_'))));
      | 
      | blocks = find_system(gcs, 'SearchDepth', 1, 'Type', 'Block');
      | 
      | for k = 1:length(blocks)
      |     if contains(extractAfter(blocks{k,1}, '/'), 'Source')
      |         set_param(blocks{k}, 'BackgroundColor', '[0.929000, 0.490000, 0.439000]');
      |     end
      | end
      settings: NameChangeFcn=|
      | Component_Name = get_param(gcb, 'Name');
      | old_ID = get_param(gcb, 'Bus_ID');
      | 
      | pattern = '_\d+';
      | match = regexp(Component_Name, pattern, 'match');
      | 
      | if ~isempty(match)
      |     if ~isequal(old_ID, num2str(strtrim(extractAfter(Component_Name, '_'))))
      |         set_param(gcb, 'Bus_ID', num2str(strtrim(extractAfter(Component_Name, '_'))));
      |     end
      | else
      |     newName = [Component_Name '_' old_ID];
      |     set_param(gcb, 'Name', newName);
      | end
      | 
      | if ~isequal(old_ID, get_param(gcb, 'Bus_ID'))
      | 
      |     data = get_param(gcb, 'PortConnectivity');
      |     for i = 1:numel(data)
      |         sourceHandle = data(i,1).SrcBlock;
      |         if ~isempty(sourceHandle) && sourceHandle ~= -1
      |             sourceParams = get_param(sourceHandle, 'DialogParameters');
      |             fn = fieldnames(sourceParams);
      |             if contains(fn{2}, 'Source')
      |                 Bus_ID = get_param(gcb, 'Bus_ID');
      |                 set_param(sourceHandle, 'Source_ID', Bus_ID);
      |             end
      |         end
      |     end
      | 
      |     blocks = find_system(gcs, 'SearchDepth', 1, 'Type', 'Block');
      | 
      |     for k = 1:length(blocks)
      |         if contains(extractAfter(blocks{k,1}, '/'), 'Source')
      |             set_param(blocks{k}, 'BackgroundColor', '[0.929000, 0.490000, 0.439000]');
      |         end
      |     end
      | 
      | end
      settings: PreDeleteFcn=|
      | blocks = find_system(gcs, 'SearchDepth', 1, 'Type', 'Block');
      | 
      | for k = 1:length(blocks)
      |     if contains(extractAfter(blocks{k,1}, '/'), 'Source')
      |         set_param(blocks{k}, 'BackgroundColor', '[0.929000, 0.490000, 0.439000]');
      |     end
      | end
  Bus_29 : MATLAB Function  TreatAsAtomicUnit=on  mask{MyInitialization=0, Bus_ID=29, Fault_flag=1}
      mask prompts: Bus_ID "Bus ID"; Fault_flag "Fault flag"
      settings: CopyFcn=|
      | Component_Name = get_param(gcb, 'Name');
      | set_param(gcb, 'Bus_ID', num2str(strtrim(extractAfter(Component_Name, '_'))));
      | 
      | blocks = find_system(gcs, 'SearchDepth', 1, 'Type', 'Block');
      | 
      | for k = 1:length(blocks)
      |     if contains(extractAfter(blocks{k,1}, '/'), 'Source')
      |         set_param(blocks{k}, 'BackgroundColor', '[0.929000, 0.490000, 0.439000]');
      |     end
      | end
      settings: NameChangeFcn=|
      | Component_Name = get_param(gcb, 'Name');
      | old_ID = get_param(gcb, 'Bus_ID');
      | 
      | pattern = '_\d+';
      | match = regexp(Component_Name, pattern, 'match');
      | 
      | if ~isempty(match)
      |     if ~isequal(old_ID, num2str(strtrim(extractAfter(Component_Name, '_'))))
      |         set_param(gcb, 'Bus_ID', num2str(strtrim(extractAfter(Component_Name, '_'))));
      |     end
      | else
      |     newName = [Component_Name '_' old_ID];
      |     set_param(gcb, 'Name', newName);
      | end
      | 
      | if ~isequal(old_ID, get_param(gcb, 'Bus_ID'))
      | 
      |     data = get_param(gcb, 'PortConnectivity');
      |     for i = 1:numel(data)
      |         sourceHandle = data(i,1).SrcBlock;
      |         if ~isempty(sourceHandle) && sourceHandle ~= -1
      |             sourceParams = get_param(sourceHandle, 'DialogParameters');
      |             fn = fieldnames(sourceParams);
      |             if contains(fn{2}, 'Source')
      |                 Bus_ID = get_param(gcb, 'Bus_ID');
      |                 set_param(sourceHandle, 'Source_ID', Bus_ID);
      |             end
      |         end
      |     end
      | 
      |     blocks = find_system(gcs, 'SearchDepth', 1, 'Type', 'Block');
      | 
      |     for k = 1:length(blocks)
      |         if contains(extractAfter(blocks{k,1}, '/'), 'Source')
      |             set_param(blocks{k}, 'BackgroundColor', '[0.929000, 0.490000, 0.439000]');
      |         end
      |     end
      | 
      | end
      settings: PreDeleteFcn=|
      | blocks = find_system(gcs, 'SearchDepth', 1, 'Type', 'Block');
      | 
      | for k = 1:length(blocks)
      |     if contains(extractAfter(blocks{k,1}, '/'), 'Source')
      |         set_param(blocks{k}, 'BackgroundColor', '[0.929000, 0.490000, 0.439000]');
      |     end
      | end
  Bus_3 : MATLAB Function  TreatAsAtomicUnit=on  mask{MyInitialization=0, Bus_ID=3, Fault_flag=1}
      mask prompts: Bus_ID "Bus ID"; Fault_flag "Fault flag"
      settings: CopyFcn=|
      | Component_Name = get_param(gcb, 'Name');
      | set_param(gcb, 'Bus_ID', num2str(strtrim(extractAfter(Component_Name, '_'))));
      | 
      | blocks = find_system(gcs, 'SearchDepth', 1, 'Type', 'Block');
      | 
      | for k = 1:length(blocks)
      |     if contains(extractAfter(blocks{k,1}, '/'), 'Source')
      |         set_param(blocks{k}, 'BackgroundColor', '[0.929000, 0.490000, 0.439000]');
      |     end
      | end
      settings: NameChangeFcn=|
      | Component_Name = get_param(gcb, 'Name');
      | old_ID = get_param(gcb, 'Bus_ID');
      | 
      | pattern = '_\d+';
      | match = regexp(Component_Name, pattern, 'match');
      | 
      | if ~isempty(match)
      |     if ~isequal(old_ID, num2str(strtrim(extractAfter(Component_Name, '_'))))
      |         set_param(gcb, 'Bus_ID', num2str(strtrim(extractAfter(Component_Name, '_'))));
      |     end
      | else
      |     newName = [Component_Name '_' old_ID];
      |     set_param(gcb, 'Name', newName);
      | end
      | 
      | if ~isequal(old_ID, get_param(gcb, 'Bus_ID'))
      | 
      |     data = get_param(gcb, 'PortConnectivity');
      |     for i = 1:numel(data)
      |         sourceHandle = data(i,1).SrcBlock;
      |         if ~isempty(sourceHandle) && sourceHandle ~= -1
      |             sourceParams = get_param(sourceHandle, 'DialogParameters');
      |             fn = fieldnames(sourceParams);
      |             if contains(fn{2}, 'Source')
      |                 Bus_ID = get_param(gcb, 'Bus_ID');
      |                 set_param(sourceHandle, 'Source_ID', Bus_ID);
      |             end
      |         end
      |     end
      | 
      |     blocks = find_system(gcs, 'SearchDepth', 1, 'Type', 'Block');
      | 
      |     for k = 1:length(blocks)
      |         if contains(extractAfter(blocks{k,1}, '/'), 'Source')
      |             set_param(blocks{k}, 'BackgroundColor', '[0.929000, 0.490000, 0.439000]');
      |         end
      |     end
      | 
      | end
      settings: PreDeleteFcn=|
      | blocks = find_system(gcs, 'SearchDepth', 1, 'Type', 'Block');
      | 
      | for k = 1:length(blocks)
      |     if contains(extractAfter(blocks{k,1}, '/'), 'Source')
      |         set_param(blocks{k}, 'BackgroundColor', '[0.929000, 0.490000, 0.439000]');
      |     end
      | end
  Bus_30 : MATLAB Function  TreatAsAtomicUnit=on  mask{MyInitialization=0, Bus_ID=30, Fault_flag=1}
      mask prompts: Bus_ID "Bus ID"; Fault_flag "Fault flag"
      settings: CopyFcn=|
      | Component_Name = get_param(gcb, 'Name');
      | set_param(gcb, 'Bus_ID', num2str(strtrim(extractAfter(Component_Name, '_'))));
      | 
      | blocks = find_system(gcs, 'SearchDepth', 1, 'Type', 'Block');
      | 
      | for k = 1:length(blocks)
      |     if contains(extractAfter(blocks{k,1}, '/'), 'Source')
      |         set_param(blocks{k}, 'BackgroundColor', '[0.929000, 0.490000, 0.439000]');
      |     end
      | end
      settings: NameChangeFcn=|
      | Component_Name = get_param(gcb, 'Name');
      | old_ID = get_param(gcb, 'Bus_ID');
      | 
      | pattern = '_\d+';
      | match = regexp(Component_Name, pattern, 'match');
      | 
      | if ~isempty(match)
      |     if ~isequal(old_ID, num2str(strtrim(extractAfter(Component_Name, '_'))))
      |         set_param(gcb, 'Bus_ID', num2str(strtrim(extractAfter(Component_Name, '_'))));
      |     end
      | else
      |     newName = [Component_Name '_' old_ID];
      |     set_param(gcb, 'Name', newName);
      | end
      | 
      | if ~isequal(old_ID, get_param(gcb, 'Bus_ID'))
      | 
      |     data = get_param(gcb, 'PortConnectivity');
      |     for i = 1:numel(data)
      |         sourceHandle = data(i,1).SrcBlock;
      |         if ~isempty(sourceHandle) && sourceHandle ~= -1
      |             sourceParams = get_param(sourceHandle, 'DialogParameters');
      |             fn = fieldnames(sourceParams);
      |             if contains(fn{2}, 'Source')
      |                 Bus_ID = get_param(gcb, 'Bus_ID');
      |                 set_param(sourceHandle, 'Source_ID', Bus_ID);
      |             end
      |         end
      |     end
      | 
      |     blocks = find_system(gcs, 'SearchDepth', 1, 'Type', 'Block');
      | 
      |     for k = 1:length(blocks)
      |         if contains(extractAfter(blocks{k,1}, '/'), 'Source')
      |             set_param(blocks{k}, 'BackgroundColor', '[0.929000, 0.490000, 0.439000]');
      |         end
      |     end
      | 
      | end
      settings: PreDeleteFcn=|
      | blocks = find_system(gcs, 'SearchDepth', 1, 'Type', 'Block');
      | 
      | for k = 1:length(blocks)
      |     if contains(extractAfter(blocks{k,1}, '/'), 'Source')
      |         set_param(blocks{k}, 'BackgroundColor', '[0.929000, 0.490000, 0.439000]');
      |     end
      | end
  Bus_4 : MATLAB Function  TreatAsAtomicUnit=on  mask{MyInitialization=0, Bus_ID=4, Fault_flag=1}
      mask prompts: Bus_ID "Bus ID"; Fault_flag "Fault flag"
      settings: CopyFcn=|
      | Component_Name = get_param(gcb, 'Name');
      | set_param(gcb, 'Bus_ID', num2str(strtrim(extractAfter(Component_Name, '_'))));
      | 
      | blocks = find_system(gcs, 'SearchDepth', 1, 'Type', 'Block');
      | 
      | for k = 1:length(blocks)
      |     if contains(extractAfter(blocks{k,1}, '/'), 'Source')
      |         set_param(blocks{k}, 'BackgroundColor', '[0.929000, 0.490000, 0.439000]');
      |     end
      | end
      settings: NameChangeFcn=|
      | Component_Name = get_param(gcb, 'Name');
      | old_ID = get_param(gcb, 'Bus_ID');
      | 
      | pattern = '_\d+';
      | match = regexp(Component_Name, pattern, 'match');
      | 
      | if ~isempty(match)
      |     if ~isequal(old_ID, num2str(strtrim(extractAfter(Component_Name, '_'))))
      |         set_param(gcb, 'Bus_ID', num2str(strtrim(extractAfter(Component_Name, '_'))));
      |     end
      | else
      |     newName = [Component_Name '_' old_ID];
      |     set_param(gcb, 'Name', newName);
      | end
      | 
      | if ~isequal(old_ID, get_param(gcb, 'Bus_ID'))
      | 
      |     data = get_param(gcb, 'PortConnectivity');
      |     for i = 1:numel(data)
      |         sourceHandle = data(i,1).SrcBlock;
      |         if ~isempty(sourceHandle) && sourceHandle ~= -1
      |             sourceParams = get_param(sourceHandle, 'DialogParameters');
      |             fn = fieldnames(sourceParams);
      |             if contains(fn{2}, 'Source')
      |                 Bus_ID = get_param(gcb, 'Bus_ID');
      |                 set_param(sourceHandle, 'Source_ID', Bus_ID);
      |             end
      |         end
      |     end
      | 
      |     blocks = find_system(gcs, 'SearchDepth', 1, 'Type', 'Block');
      | 
      |     for k = 1:length(blocks)
      |         if contains(extractAfter(blocks{k,1}, '/'), 'Source')
      |             set_param(blocks{k}, 'BackgroundColor', '[0.929000, 0.490000, 0.439000]');
      |         end
      |     end
      | 
      | end
      settings: PreDeleteFcn=|
      | blocks = find_system(gcs, 'SearchDepth', 1, 'Type', 'Block');
      | 
      | for k = 1:length(blocks)
      |     if contains(extractAfter(blocks{k,1}, '/'), 'Source')
      |         set_param(blocks{k}, 'BackgroundColor', '[0.929000, 0.490000, 0.439000]');
      |     end
      | end
  Bus_5 : MATLAB Function  TreatAsAtomicUnit=on  mask{MyInitialization=0, Bus_ID=5, Fault_flag=1}
      mask prompts: Bus_ID "Bus ID"; Fault_flag "Fault flag"
      settings: CopyFcn=|
      | Component_Name = get_param(gcb, 'Name');
      | set_param(gcb, 'Bus_ID', num2str(strtrim(extractAfter(Component_Name, '_'))));
      | 
      | blocks = find_system(gcs, 'SearchDepth', 1, 'Type', 'Block');
      | 
      | for k = 1:length(blocks)
      |     if contains(extractAfter(blocks{k,1}, '/'), 'Source')
      |         set_param(blocks{k}, 'BackgroundColor', '[0.929000, 0.490000, 0.439000]');
      |     end
      | end
      settings: NameChangeFcn=|
      | Component_Name = get_param(gcb, 'Name');
      | old_ID = get_param(gcb, 'Bus_ID');
      | 
      | pattern = '_\d+';
      | match = regexp(Component_Name, pattern, 'match');
      | 
      | if ~isempty(match)
      |     if ~isequal(old_ID, num2str(strtrim(extractAfter(Component_Name, '_'))))
      |         set_param(gcb, 'Bus_ID', num2str(strtrim(extractAfter(Component_Name, '_'))));
      |     end
      | else
      |     newName = [Component_Name '_' old_ID];
      |     set_param(gcb, 'Name', newName);
      | end
      | 
      | if ~isequal(old_ID, get_param(gcb, 'Bus_ID'))
      | 
      |     data = get_param(gcb, 'PortConnectivity');
      |     for i = 1:numel(data)
      |         sourceHandle = data(i,1).SrcBlock;
      |         if ~isempty(sourceHandle) && sourceHandle ~= -1
      |             sourceParams = get_param(sourceHandle, 'DialogParameters');
      |             fn = fieldnames(sourceParams);
      |             if contains(fn{2}, 'Source')
      |                 Bus_ID = get_param(gcb, 'Bus_ID');
      |                 set_param(sourceHandle, 'Source_ID', Bus_ID);
      |             end
      |         end
      |     end
      | 
      |     blocks = find_system(gcs, 'SearchDepth', 1, 'Type', 'Block');
      | 
      |     for k = 1:length(blocks)
      |         if contains(extractAfter(blocks{k,1}, '/'), 'Source')
      |             set_param(blocks{k}, 'BackgroundColor', '[0.929000, 0.490000, 0.439000]');
      |         end
      |     end
      | 
      | end
      settings: PreDeleteFcn=|
      | blocks = find_system(gcs, 'SearchDepth', 1, 'Type', 'Block');
      | 
      | for k = 1:length(blocks)
      |     if contains(extractAfter(blocks{k,1}, '/'), 'Source')
      |         set_param(blocks{k}, 'BackgroundColor', '[0.929000, 0.490000, 0.439000]');
      |     end
      | end
  Bus_6 : MATLAB Function  TreatAsAtomicUnit=on  mask{MyInitialization=0, Bus_ID=6, Fault_flag=1}
      mask prompts: Bus_ID "Bus ID"; Fault_flag "Fault flag"
      settings: CopyFcn=|
      | Component_Name = get_param(gcb, 'Name');
      | set_param(gcb, 'Bus_ID', num2str(strtrim(extractAfter(Component_Name, '_'))));
      | 
      | blocks = find_system(gcs, 'SearchDepth', 1, 'Type', 'Block');
      | 
      | for k = 1:length(blocks)
      |     if contains(extractAfter(blocks{k,1}, '/'), 'Source')
      |         set_param(blocks{k}, 'BackgroundColor', '[0.929000, 0.490000, 0.439000]');
      |     end
      | end
      settings: NameChangeFcn=|
      | Component_Name = get_param(gcb, 'Name');
      | old_ID = get_param(gcb, 'Bus_ID');
      | 
      | pattern = '_\d+';
      | match = regexp(Component_Name, pattern, 'match');
      | 
      | if ~isempty(match)
      |     if ~isequal(old_ID, num2str(strtrim(extractAfter(Component_Name, '_'))))
      |         set_param(gcb, 'Bus_ID', num2str(strtrim(extractAfter(Component_Name, '_'))));
      |     end
      | else
      |     newName = [Component_Name '_' old_ID];
      |     set_param(gcb, 'Name', newName);
      | end
      | 
      | if ~isequal(old_ID, get_param(gcb, 'Bus_ID'))
      | 
      |     data = get_param(gcb, 'PortConnectivity');
      |     for i = 1:numel(data)
      |         sourceHandle = data(i,1).SrcBlock;
      |         if ~isempty(sourceHandle) && sourceHandle ~= -1
      |             sourceParams = get_param(sourceHandle, 'DialogParameters');
      |             fn = fieldnames(sourceParams);
      |             if contains(fn{2}, 'Source')
      |                 Bus_ID = get_param(gcb, 'Bus_ID');
      |                 set_param(sourceHandle, 'Source_ID', Bus_ID);
      |             end
      |         end
      |     end
      | 
      |     blocks = find_system(gcs, 'SearchDepth', 1, 'Type', 'Block');
      | 
      |     for k = 1:length(blocks)
      |         if contains(extractAfter(blocks{k,1}, '/'), 'Source')
      |             set_param(blocks{k}, 'BackgroundColor', '[0.929000, 0.490000, 0.439000]');
      |         end
      |     end
      | 
      | end
      settings: PreDeleteFcn=|
      | blocks = find_system(gcs, 'SearchDepth', 1, 'Type', 'Block');
      | 
      | for k = 1:length(blocks)
      |     if contains(extractAfter(blocks{k,1}, '/'), 'Source')
      |         set_param(blocks{k}, 'BackgroundColor', '[0.929000, 0.490000, 0.439000]');
      |     end
      | end
  Bus_7 : MATLAB Function  TreatAsAtomicUnit=on  mask{MyInitialization=0, Bus_ID=7, Fault_flag=1}
      mask prompts: Bus_ID "Bus ID"; Fault_flag "Fault flag"
      settings: CopyFcn=|
      | Component_Name = get_param(gcb, 'Name');
      | set_param(gcb, 'Bus_ID', num2str(strtrim(extractAfter(Component_Name, '_'))));
      | 
      | blocks = find_system(gcs, 'SearchDepth', 1, 'Type', 'Block');
      | 
      | for k = 1:length(blocks)
      |     if contains(extractAfter(blocks{k,1}, '/'), 'Source')
      |         set_param(blocks{k}, 'BackgroundColor', '[0.929000, 0.490000, 0.439000]');
      |     end
      | end
      settings: NameChangeFcn=|
      | Component_Name = get_param(gcb, 'Name');
      | old_ID = get_param(gcb, 'Bus_ID');
      | 
      | pattern = '_\d+';
      | match = regexp(Component_Name, pattern, 'match');
      | 
      | if ~isempty(match)
      |     if ~isequal(old_ID, num2str(strtrim(extractAfter(Component_Name, '_'))))
      |         set_param(gcb, 'Bus_ID', num2str(strtrim(extractAfter(Component_Name, '_'))));
      |     end
      | else
      |     newName = [Component_Name '_' old_ID];
      |     set_param(gcb, 'Name', newName);
      | end
      | 
      | if ~isequal(old_ID, get_param(gcb, 'Bus_ID'))
      | 
      |     data = get_param(gcb, 'PortConnectivity');
      |     for i = 1:numel(data)
      |         sourceHandle = data(i,1).SrcBlock;
      |         if ~isempty(sourceHandle) && sourceHandle ~= -1
      |             sourceParams = get_param(sourceHandle, 'DialogParameters');
      |             fn = fieldnames(sourceParams);
      |             if contains(fn{2}, 'Source')
      |                 Bus_ID = get_param(gcb, 'Bus_ID');
      |                 set_param(sourceHandle, 'Source_ID', Bus_ID);
      |             end
      |         end
      |     end
      | 
      |     blocks = find_system(gcs, 'SearchDepth', 1, 'Type', 'Block');
      | 
      |     for k = 1:length(blocks)
      |         if contains(extractAfter(blocks{k,1}, '/'), 'Source')
      |             set_param(blocks{k}, 'BackgroundColor', '[0.929000, 0.490000, 0.439000]');
      |         end
      |     end
      | 
      | end
      settings: PreDeleteFcn=|
      | blocks = find_system(gcs, 'SearchDepth', 1, 'Type', 'Block');
      | 
      | for k = 1:length(blocks)
      |     if contains(extractAfter(blocks{k,1}, '/'), 'Source')
      |         set_param(blocks{k}, 'BackgroundColor', '[0.929000, 0.490000, 0.439000]');
      |     end
      | end
  Bus_8 : MATLAB Function  TreatAsAtomicUnit=on  mask{MyInitialization=0, Bus_ID=8, Fault_flag=1}
      mask prompts: Bus_ID "Bus ID"; Fault_flag "Fault flag"
      settings: CopyFcn=|
      | Component_Name = get_param(gcb, 'Name');
      | set_param(gcb, 'Bus_ID', num2str(strtrim(extractAfter(Component_Name, '_'))));
      | 
      | blocks = find_system(gcs, 'SearchDepth', 1, 'Type', 'Block');
      | 
      | for k = 1:length(blocks)
      |     if contains(extractAfter(blocks{k,1}, '/'), 'Source')
      |         set_param(blocks{k}, 'BackgroundColor', '[0.929000, 0.490000, 0.439000]');
      |     end
      | end
      settings: NameChangeFcn=|
      | Component_Name = get_param(gcb, 'Name');
      | old_ID = get_param(gcb, 'Bus_ID');
      | 
      | pattern = '_\d+';
      | match = regexp(Component_Name, pattern, 'match');
      | 
      | if ~isempty(match)
      |     if ~isequal(old_ID, num2str(strtrim(extractAfter(Component_Name, '_'))))
      |         set_param(gcb, 'Bus_ID', num2str(strtrim(extractAfter(Component_Name, '_'))));
      |     end
      | else
      |     newName = [Component_Name '_' old_ID];
      |     set_param(gcb, 'Name', newName);
      | end
      | 
      | if ~isequal(old_ID, get_param(gcb, 'Bus_ID'))
      | 
      |     data = get_param(gcb, 'PortConnectivity');
      |     for i = 1:numel(data)
      |         sourceHandle = data(i,1).SrcBlock;
      |         if ~isempty(sourceHandle) && sourceHandle ~= -1
      |             sourceParams = get_param(sourceHandle, 'DialogParameters');
      |             fn = fieldnames(sourceParams);
      |             if contains(fn{2}, 'Source')
      |                 Bus_ID = get_param(gcb, 'Bus_ID');
      |                 set_param(sourceHandle, 'Source_ID', Bus_ID);
      |             end
      |         end
      |     end
      | 
      |     blocks = find_system(gcs, 'SearchDepth', 1, 'Type', 'Block');
      | 
      |     for k = 1:length(blocks)
      |         if contains(extractAfter(blocks{k,1}, '/'), 'Source')
      |             set_param(blocks{k}, 'BackgroundColor', '[0.929000, 0.490000, 0.439000]');
      |         end
      |     end
      | 
      | end
      settings: PreDeleteFcn=|
      | blocks = find_system(gcs, 'SearchDepth', 1, 'Type', 'Block');
      | 
      | for k = 1:length(blocks)
      |     if contains(extractAfter(blocks{k,1}, '/'), 'Source')
      |         set_param(blocks{k}, 'BackgroundColor', '[0.929000, 0.490000, 0.439000]');
      |     end
      | end
  Bus_9 : MATLAB Function  TreatAsAtomicUnit=on  mask{MyInitialization=0, Bus_ID=9, Fault_flag=1}
      mask prompts: Bus_ID "Bus ID"; Fault_flag "Fault flag"
      settings: CopyFcn=|
      | Component_Name = get_param(gcb, 'Name');
      | set_param(gcb, 'Bus_ID', num2str(strtrim(extractAfter(Component_Name, '_'))));
      | 
      | blocks = find_system(gcs, 'SearchDepth', 1, 'Type', 'Block');
      | 
      | for k = 1:length(blocks)
      |     if contains(extractAfter(blocks{k,1}, '/'), 'Source')
      |         set_param(blocks{k}, 'BackgroundColor', '[0.929000, 0.490000, 0.439000]');
      |     end
      | end
      settings: NameChangeFcn=|
      | Component_Name = get_param(gcb, 'Name');
      | old_ID = get_param(gcb, 'Bus_ID');
      | 
      | pattern = '_\d+';
      | match = regexp(Component_Name, pattern, 'match');
      | 
      | if ~isempty(match)
      |     if ~isequal(old_ID, num2str(strtrim(extractAfter(Component_Name, '_'))))
      |         set_param(gcb, 'Bus_ID', num2str(strtrim(extractAfter(Component_Name, '_'))));
      |     end
      | else
      |     newName = [Component_Name '_' old_ID];
      |     set_param(gcb, 'Name', newName);
      | end
      | 
      | if ~isequal(old_ID, get_param(gcb, 'Bus_ID'))
      | 
      |     data = get_param(gcb, 'PortConnectivity');
      |     for i = 1:numel(data)
      |         sourceHandle = data(i,1).SrcBlock;
      |         if ~isempty(sourceHandle) && sourceHandle ~= -1
      |             sourceParams = get_param(sourceHandle, 'DialogParameters');
      |             fn = fieldnames(sourceParams);
      |             if contains(fn{2}, 'Source')
      |                 Bus_ID = get_param(gcb, 'Bus_ID');
      |                 set_param(sourceHandle, 'Source_ID', Bus_ID);
      |             end
      |         end
      |     end
      | 
      |     blocks = find_system(gcs, 'SearchDepth', 1, 'Type', 'Block');
      | 
      |     for k = 1:length(blocks)
      |         if contains(extractAfter(blocks{k,1}, '/'), 'Source')
      |             set_param(blocks{k}, 'BackgroundColor', '[0.929000, 0.490000, 0.439000]');
      |         end
      |     end
      | 
      | end
      settings: PreDeleteFcn=|
      | blocks = find_system(gcs, 'SearchDepth', 1, 'Type', 'Block');
      | 
      | for k = 1:length(blocks)
      |     if contains(extractAfter(blocks{k,1}, '/'), 'Source')
      |         set_param(blocks{k}, 'BackgroundColor', '[0.929000, 0.490000, 0.439000]');
      |     end
      | end
  CB_1 : ABB_UPPAAL_Library/CB_1  MyInitialization=0  CB_ID=1  Sel_Type=3  m=3  i1=360  t1=180  i2_flag=off  i2=null  t2=null  i3_flag=off  i3=null  t3=null  i7=720  t7FW=8  t7BW=8  tselFW=1  tselBW=1  Actors={ '3', '1', '1' }
      settings: SourceProductName=ABB UPPAAL Library
  CB_10 : ABB_UPPAAL_Library/CB_1  MyInitialization=0  CB_ID=10  Sel_Type=1  m=3  i1=90  t1=140  i2_flag=on  i2=180  t2=6  i3_flag=off  i3=null  t3=null  i7=null  t7FW=null  t7BW=null  tselFW=null  tselBW=null  Actors={}
      settings: SourceProductName=ABB UPPAAL Library
  CB_11 : ABB_UPPAAL_Library/CB_1  MyInitialization=0  CB_ID=11  Sel_Type=1  m=3  i1=30  t1=100  i2_flag=on  i2=60  t2=2  i3_flag=off  i3=null  t3=null  i7=null  t7FW=null  t7BW=null  tselFW=null  tselBW=null  Actors={}
      settings: SourceProductName=ABB UPPAAL Library
  CB_12 : ABB_UPPAAL_Library/CB_1  MyInitialization=0  CB_ID=12  Sel_Type=1  m=3  i1=60  t1=120  i2_flag=on  i2=120  t2=4  i3_flag=off  i3=null  t3=null  i7=null  t7FW=null  t7BW=null  tselFW=null  tselBW=null  Actors={}
      settings: SourceProductName=ABB UPPAAL Library
  CB_13 : ABB_UPPAAL_Library/CB_1  MyInitialization=0  CB_ID=13  Sel_Type=1  m=3  i1=30  t1=100  i2_flag=on  i2=60  t2=2  i3_flag=off  i3=null  t3=null  i7=null  t7FW=null  t7BW=null  tselFW=null  tselBW=null  Actors={}
      settings: SourceProductName=ABB UPPAAL Library
  CB_14 : ABB_UPPAAL_Library/CB_1  MyInitialization=0  CB_ID=14  Sel_Type=1  m=3  i1=30  t1=100  i2_flag=on  i2=60  t2=2  i3_flag=off  i3=null  t3=null  i7=null  t7FW=null  t7BW=null  tselFW=null  tselBW=null  Actors={}
      settings: SourceProductName=ABB UPPAAL Library
  CB_15 : ABB_UPPAAL_Library/CB_1  MyInitialization=0  CB_ID=15  Sel_Type=3  m=3  i1=180  t1=170  i2_flag=off  i2=null  t2=null  i3_flag=off  i3=null  t3=null  i7=360  t7FW=7  t7BW=7  tselFW=1  tselBW=1  Actors={ '8', '0', '0'; '9', '0', '0'; '10', '1', '0'; '16', '0', '1'; '23', '1', '1' }
      settings: SourceProductName=ABB UPPAAL Library
  CB_16 : ABB_UPPAAL_Library/CB_1  MyInitialization=0  CB_ID=16  Sel_Type=3  m=3  i1=360  t1=180  i2_flag=off  i2=null  t2=null  i3_flag=off  i3=null  t3=null  i7=720  t7FW=8  t7BW=8  tselFW=1  tselBW=1  Actors={ '15', '0', '1'; '23', '1', '1' }
      settings: SourceProductName=ABB UPPAAL Library
  CB_17 : ABB_UPPAAL_Library/CB_1  MyInitialization=0  CB_ID=17  Sel_Type=1  m=3  i1=90  t1=140  i2_flag=on  i2=180  t2=6  i3_flag=off  i3=null  t3=null  i7=null  t7FW=null  t7BW=null  tselFW=null  tselBW=null  Actors={}
      settings: SourceProductName=ABB UPPAAL Library
  CB_18 : ABB_UPPAAL_Library/CB_1  MyInitialization=0  CB_ID=18  Sel_Type=1  m=3  i1=30  t1=100  i2_flag=on  i2=60  t2=2  i3_flag=off  i3=null  t3=null  i7=null  t7FW=null  t7BW=null  tselFW=null  tselBW=null  Actors={}
      settings: SourceProductName=ABB UPPAAL Library
  CB_19 : ABB_UPPAAL_Library/CB_1  MyInitialization=0  CB_ID=19  Sel_Type=1  m=3  i1=60  t1=120  i2_flag=on  i2=120  t2=4  i3_flag=off  i3=null  t3=null  i7=null  t7FW=null  t7BW=null  tselFW=null  tselBW=null  Actors={}
      settings: SourceProductName=ABB UPPAAL Library
  CB_2 : ABB_UPPAAL_Library/CB_1  MyInitialization=0  CB_ID=2  Sel_Type=3  m=3  i1=360  t1=180  i2_flag=off  i2=null  t2=null  i3_flag=off  i3=null  t3=null  i7=720  t7FW=8  t7BW=8  tselFW=1  tselBW=1  Actors={ '3', '0', '1'; '4', '1', '1'; '9', '1', '1' }
      settings: SourceProductName=ABB UPPAAL Library
  CB_20 : ABB_UPPAAL_Library/CB_1  MyInitialization=0  CB_ID=20  Sel_Type=1  m=3  i1=30  t1=100  i2_flag=on  i2=60  t2=2  i3_flag=off  i3=null  t3=null  i7=null  t7FW=null  t7BW=null  tselFW=null  tselBW=null  Actors={}
      settings: SourceProductName=ABB UPPAAL Library
  CB_21 : ABB_UPPAAL_Library/CB_1  MyInitialization=0  CB_ID=21  Sel_Type=1  m=3  i1=30  t1=100  i2_flag=on  i2=60  t2=2  i3_flag=off  i3=null  t3=null  i7=null  t7FW=null  t7BW=null  tselFW=null  tselBW=null  Actors={}
      settings: SourceProductName=ABB UPPAAL Library
  CB_22 : ABB_UPPAAL_Library/CB_1  MyInitialization=0  CB_ID=22  Sel_Type=3  m=3  i1=360  t1=180  i2_flag=off  i2=null  t2=null  i3_flag=off  i3=null  t3=null  i7=720  t7FW=8  t7BW=8  tselFW=1  tselBW=1  Actors={ '23', '0', '1'; '24', '1', '1'; '29', '1', '1' }
      settings: SourceProductName=ABB UPPAAL Library
  CB_23 : ABB_UPPAAL_Library/CB_1  MyInitialization=0  CB_ID=23  Sel_Type=3  m=3  i1=180  t1=170  i2_flag=on  i2=360  t2=null  i3_flag=off  i3=null  t3=null  i7=360  t7FW=6  t7BW=6  tselFW=1  tselBW=1  Actors={ '15', '0', '0'; '16', '0', '0'; '22', '0', '1'; '24', '1', '1'; '29', '1', '1' }
      settings: SourceProductName=ABB UPPAAL Library
  CB_24 : ABB_UPPAAL_Library/CB_1  MyInitialization=0  CB_ID=24  Sel_Type=1  m=3  i1=90  t1=120  i2_flag=on  i2=180  t2=4  i3_flag=off  i3=null  t3=null  i7=null  t7FW=null  t7BW=null  tselFW=null  tselBW=null  Actors={}
      settings: SourceProductName=ABB UPPAAL Library
  CB_25 : ABB_UPPAAL_Library/CB_1  MyInitialization=0  CB_ID=25  Sel_Type=1  m=3  i1=30  t1=100  i2_flag=on  i2=60  t2=2  i3_flag=off  i3=null  t3=null  i7=null  t7FW=null  t7BW=null  tselFW=null  tselBW=null  Actors={}
      settings: SourceProductName=ABB UPPAAL Library
  CB_26 : ABB_UPPAAL_Library/CB_1  MyInitialization=0  CB_ID=26  Sel_Type=1  m=3  i1=30  t1=100  i2_flag=on  i2=60  t2=2  i3_flag=off  i3=null  t3=null  i7=null  t7FW=null  t7BW=null  tselFW=null  tselBW=null  Actors={}
      settings: SourceProductName=ABB UPPAAL Library
  CB_27 : ABB_UPPAAL_Library/CB_1  MyInitialization=0  CB_ID=27  Sel_Type=1  m=3  i1=30  t1=100  i2_flag=on  i2=60  t2=2  i3_flag=off  i3=null  t3=null  i7=null  t7FW=null  t7BW=null  tselFW=null  tselBW=null  Actors={}
      settings: SourceProductName=ABB UPPAAL Library
  CB_28 : ABB_UPPAAL_Library/CB_1  MyInitialization=0  CB_ID=28  Sel_Type=3  m=3  i1=360  t1=180  i2_flag=off  i2=null  t2=null  i3_flag=off  i3=null  t3=null  i7=720  t7FW=8  t7BW=8  tselFW=1  tselBW=1  Actors={ '17', '1', '1'; '29', '0', '1' }
      settings: SourceProductName=ABB UPPAAL Library
  CB_29 : ABB_UPPAAL_Library/CB_1  MyInitialization=0  CB_ID=29  Sel_Type=3  m=3  i1=270  t1=170  i2_flag=off  i2=null  t2=null  i3_flag=off  i3=null  t3=null  i7=540  t7FW=5  t7BW=5  tselFW=1  tselBW=1  Actors={ '22', '0', '0'; '23', '0', '0'; '24', '1', '0'; '17', '1', '1'; '28', '0', '1' }
      settings: SourceProductName=ABB UPPAAL Library
  CB_3 : ABB_UPPAAL_Library/CB_1  MyInitialization=0  CB_ID=3  Sel_Type=3  m=3  i1=360  t1=170  i2_flag=off  i2=null  t2=null  i3_flag=off  i3=null  t3=null  i7=720  t7FW=7  t7BW=7  tselFW=1  tselBW=1  Actors={ '1', '0', '0'; '2', '0', '1'; '4', '1', '1'; '9', '1', '1' }
      settings: SourceProductName=ABB UPPAAL Library
  CB_4 : ABB_UPPAAL_Library/CB_1  MyInitialization=0  CB_ID=4  Sel_Type=1  m=3  i1=90  t1=120  i2_flag=on  i2=180  t2=4  i3_flag=off  i3=null  t3=null  i7=null  t7FW=null  t7BW=null  tselFW=null  tselBW=null  Actors={}
      settings: SourceProductName=ABB UPPAAL Library
  CB_5 : ABB_UPPAAL_Library/CB_1  MyInitialization=0  CB_ID=5  Sel_Type=1  m=3  i1=30  t1=100  i2_flag=on  i2=60  t2=2  i3_flag=off  i3=null  t3=null  i7=null  t7FW=null  t7BW=null  tselFW=null  tselBW=null  Actors={}
      settings: SourceProductName=ABB UPPAAL Library
  CB_6 : ABB_UPPAAL_Library/CB_1  MyInitialization=0  CB_ID=6  Sel_Type=1  m=3  i1=30  t1=100  i2_flag=on  i2=60  t2=2  i3_flag=off  i3=null  t3=null  i7=null  t7FW=null  t7BW=null  tselFW=null  tselBW=null  Actors={}
      settings: SourceProductName=ABB UPPAAL Library
  CB_7 : ABB_UPPAAL_Library/CB_1  MyInitialization=0  CB_ID=7  Sel_Type=1  m=3  i1=30  t1=100  i2_flag=on  i2=60  t2=2  i3_flag=off  i3=null  t3=null  i7=null  t7FW=null  t7BW=null  tselFW=null  tselBW=null  Actors={}
      settings: SourceProductName=ABB UPPAAL Library
  CB_8 : ABB_UPPAAL_Library/CB_1  MyInitialization=0  CB_ID=8  Sel_Type=3  m=3  i1=360  t1=180  i2_flag=off  i2=null  t2=null  i3_flag=off  i3=null  t3=null  i7=720  t7FW=8  t7BW=8  tselFW=1  tselBW=1  Actors={ '9', '0', '1'; '10', '1', '1'; '15', '1', '1' }
      settings: SourceProductName=ABB UPPAAL Library
  CB_9 : ABB_UPPAAL_Library/CB_1  MyInitialization=0  CB_ID=9  Sel_Type=3  m=3  i1=270  t1=170  i2_flag=off  i2=null  t2=null  i3_flag=off  i3=null  t3=null  i7=540  t7FW=7  t7BW=7  tselFW=1  tselBW=1  Actors={ '2', '0', '0'; '3', '0', '0'; '4', '1', '0'; '8', '0', '1'; '10', '1', '1'; '15', '1', '1' }
      settings: SourceProductName=ABB UPPAAL Library
  Line_1 : ABB_UPPAAL_Library/Line_1  MyInitialization=0  Line_ID=1  Iioc=50  Ith=360  Fault_flag=1
      settings: SourceProductName=ABB UPPAAL Library
  Line_10 : ABB_UPPAAL_Library/Line_1  MyInitialization=0  Line_ID=10  Iioc=75  Ith=90  Fault_flag=1
      settings: SourceProductName=ABB UPPAAL Library
  Line_11 : ABB_UPPAAL_Library/Line_1  MyInitialization=0  Line_ID=11  Iioc=25  Ith=30  Fault_flag=1
      settings: SourceProductName=ABB UPPAAL Library
  Line_12 : ABB_UPPAAL_Library/Line_1  MyInitialization=0  Line_ID=12  Iioc=50  Ith=60  Fault_flag=1
      settings: SourceProductName=ABB UPPAAL Library
  Line_13 : ABB_UPPAAL_Library/Line_1  MyInitialization=0  Line_ID=13  Iioc=25  Ith=30  Fault_flag=1
      settings: SourceProductName=ABB UPPAAL Library
  Line_14 : ABB_UPPAAL_Library/Line_1  MyInitialization=0  Line_ID=14  Iioc=25  Ith=30  Fault_flag=1
      settings: SourceProductName=ABB UPPAAL Library
  Line_15 : ABB_UPPAAL_Library/Line_1  MyInitialization=0  Line_ID=15  Iioc=25  Ith=180  Fault_flag=1
      settings: SourceProductName=ABB UPPAAL Library
  Line_16 : ABB_UPPAAL_Library/Line_1  MyInitialization=0  Line_ID=16  Iioc=25  Ith=360  Fault_flag=1
      settings: SourceProductName=ABB UPPAAL Library
  Line_17 : ABB_UPPAAL_Library/Line_1  MyInitialization=0  Line_ID=17  Iioc=75  Ith=90  Fault_flag=1
      settings: SourceProductName=ABB UPPAAL Library
  Line_18 : ABB_UPPAAL_Library/Line_1  MyInitialization=0  Line_ID=18  Iioc=25  Ith=30  Fault_flag=1
      settings: SourceProductName=ABB UPPAAL Library
  Line_19 : ABB_UPPAAL_Library/Line_1  MyInitialization=0  Line_ID=19  Iioc=50  Ith=60  Fault_flag=1
      settings: SourceProductName=ABB UPPAAL Library
  Line_2 : ABB_UPPAAL_Library/Line_1  MyInitialization=0  Line_ID=2  Iioc=50  Ith=360  Fault_flag=1
      settings: SourceProductName=ABB UPPAAL Library
  Line_20 : ABB_UPPAAL_Library/Line_1  MyInitialization=0  Line_ID=20  Iioc=25  Ith=30  Fault_flag=1
      settings: SourceProductName=ABB UPPAAL Library
  Line_21 : ABB_UPPAAL_Library/Line_1  MyInitialization=0  Line_ID=21  Iioc=25  Ith=30  Fault_flag=1
      settings: SourceProductName=ABB UPPAAL Library
  Line_23 : ABB_UPPAAL_Library/Line_1  MyInitialization=0  Line_ID=23  Iioc=50  Ith=360  Fault_flag=1
      settings: SourceProductName=ABB UPPAAL Library
  Line_24 : ABB_UPPAAL_Library/Line_1  MyInitialization=0  Line_ID=24  Iioc=50  Ith=180  Fault_flag=1
      settings: SourceProductName=ABB UPPAAL Library
  Line_25 : ABB_UPPAAL_Library/Line_1  MyInitialization=0  Line_ID=25  Iioc=75  Ith=90  Fault_flag=1
      settings: SourceProductName=ABB UPPAAL Library
  Line_26 : ABB_UPPAAL_Library/Line_1  MyInitialization=0  Line_ID=26  Iioc=25  Ith=30  Fault_flag=1
      settings: SourceProductName=ABB UPPAAL Library
  Line_27 : ABB_UPPAAL_Library/Line_1  MyInitialization=0  Line_ID=27  Iioc=25  Ith=30  Fault_flag=1
      settings: SourceProductName=ABB UPPAAL Library
  Line_28 : ABB_UPPAAL_Library/Line_1  MyInitialization=0  Line_ID=28  Iioc=25  Ith=30  Fault_flag=1
      settings: SourceProductName=ABB UPPAAL Library
  Line_29 : ABB_UPPAAL_Library/Line_1  MyInitialization=0  Line_ID=29  Iioc=50  Ith=360  Fault_flag=1
      settings: SourceProductName=ABB UPPAAL Library
  Line_3 : ABB_UPPAAL_Library/Line_1  MyInitialization=0  Line_ID=3  Iioc=50  Ith=360  Fault_flag=1
      settings: SourceProductName=ABB UPPAAL Library
  Line_30 : ABB_UPPAAL_Library/Line_1  MyInitialization=0  Line_ID=30  Iioc=25  Ith=270  Fault_flag=1
      settings: SourceProductName=ABB UPPAAL Library
  Line_4 : ABB_UPPAAL_Library/Line_1  MyInitialization=0  Line_ID=4  Iioc=75  Ith=90  Fault_flag=1
      settings: SourceProductName=ABB UPPAAL Library
  Line_5 : ABB_UPPAAL_Library/Line_1  MyInitialization=0  Line_ID=5  Iioc=25  Ith=30  Fault_flag=1
      settings: SourceProductName=ABB UPPAAL Library
  Line_6 : ABB_UPPAAL_Library/Line_1  MyInitialization=0  Line_ID=6  Iioc=25  Ith=30  Fault_flag=1
      settings: SourceProductName=ABB UPPAAL Library
  Line_7 : ABB_UPPAAL_Library/Line_1  MyInitialization=0  Line_ID=7  Iioc=25  Ith=30  Fault_flag=1
      settings: SourceProductName=ABB UPPAAL Library
  Line_8 : ABB_UPPAAL_Library/Line_1  MyInitialization=0  Line_ID=8  Iioc=75  Ith=360  Fault_flag=1
      settings: SourceProductName=ABB UPPAAL Library
  Line_9 : ABB_UPPAAL_Library/Line_1  MyInitialization=0  Line_ID=9  Iioc=25  Ith=270  Fault_flag=1
      settings: SourceProductName=ABB UPPAAL Library
  Load_1 : ABB_UPPAAL_Library/Load_1  MyInitialization=0  Load_ID=1
      settings: SourceProductName=ABB UPPAAL Library
  Load_10 : ABB_UPPAAL_Library/Load_1  MyInitialization=0  Load_ID=10
      settings: SourceProductName=ABB UPPAAL Library
  Load_11 : ABB_UPPAAL_Library/Load_1  MyInitialization=0  Load_ID=11
      settings: SourceProductName=ABB UPPAAL Library
  Load_12 : ABB_UPPAAL_Library/Load_1  MyInitialization=0  Load_ID=12
      settings: SourceProductName=ABB UPPAAL Library
  Load_2 : ABB_UPPAAL_Library/Load_1  MyInitialization=0  Load_ID=2
      settings: SourceProductName=ABB UPPAAL Library
  Load_3 : ABB_UPPAAL_Library/Load_1  MyInitialization=0  Load_ID=3
      settings: SourceProductName=ABB UPPAAL Library
  Load_4 : ABB_UPPAAL_Library/Load_1  MyInitialization=0  Load_ID=4
      settings: SourceProductName=ABB UPPAAL Library
  Load_5 : ABB_UPPAAL_Library/Load_1  MyInitialization=0  Load_ID=5
      settings: SourceProductName=ABB UPPAAL Library
  Load_6 : ABB_UPPAAL_Library/Load_1  MyInitialization=0  Load_ID=6
      settings: SourceProductName=ABB UPPAAL Library
  Load_7 : ABB_UPPAAL_Library/Load_1  MyInitialization=0  Load_ID=7
      settings: SourceProductName=ABB UPPAAL Library
  Load_8 : ABB_UPPAAL_Library/Load_1  MyInitialization=0  Load_ID=8
      settings: SourceProductName=ABB UPPAAL Library
  Load_9 : ABB_UPPAAL_Library/Load_1  MyInitialization=0  Load_ID=9
      settings: SourceProductName=ABB UPPAAL Library
  Source_1 : ABB_UPPAAL_Library/Source_1  MyInitialization=0  Source_ID=1  Lines_Isc={ '1', '834'; '2', '834'; '3', '834'; '4', '1250'; '5', '417'; '6', '417'; '7', '417'; '8', '1250'; '9', '417'; '10', '1250'; '11', '417'; '12', '834'; '13', '417'; '14', '417'; '15', '417'; '16', '417'; '17', '1250'; '18', '417'; '19', '834'; '20', '417'; '21', '417'; '23', '834'; '24', '834'; '25', '1250'; '26', '417'; '27', '417'; '28', '417'; '29', '834'; '30', '417' }  Buses_Isc={ '1', '834'; '2', '834'; '3', '834'; '4', '834'; '5', '1250'; '6', '417'; '7', '417'; '8', '417'; '9', '1250'; '10', '1250'; '11', '1250'; '12', '417'; '13', '834'; '14', '417'; '15', '417'; '16', '417'; '17', '834'; '18', '1250'; '19', '417'; '20', '834'; '21', '417'; '22', '417'; '23', '834'; '24', '417'; '25', '834'; '26', '1250'; '27', '417'; '28', '417'; '29', '417'; '30', '834' }
      settings: SourceProductName=ABB UPPAAL Library
  Source_16 : ABB_UPPAAL_Library/Source_1  MyInitialization=0  Source_ID=16  Lines_Isc={ '1', '417'; '2', '417'; '3', '417'; '4', '625'; '5', '209'; '6', '209'; '7', '209'; '8', '625'; '9', '625'; '10', '625'; '11', '209'; '12', '417'; '13', '209'; '14', '209'; '15', '209'; '16', '625'; '17', '625'; '18', '209'; '19', '417'; '20', '209'; '21', '209'; '23', '417'; '24', '417'; '25', '625'; '26', '209'; '27', '209'; '28', '209'; '29', '417'; '30', '625' }  Buses_Isc={ '1', '417'; '2', '417'; '3', '417'; '4', '417'; '5', '625'; '6', '209'; '7', '209'; '8', '209'; '9', '625'; '10', '625'; '11', '625'; '12', '209'; '13', '417'; '14', '209'; '15', '209'; '16', '209'; '17', '417'; '18', '625'; '19', '209'; '20', '417'; '21', '209'; '22', '209'; '23', '417'; '24', '209'; '25', '417'; '26', '625'; '27', '209'; '28', '209'; '29', '209'; '30', '417' }
      settings: SourceProductName=ABB UPPAAL Library
  Source_2 : ABB_UPPAAL_Library/Source_1  MyInitialization=0  Source_ID=2  Lines_Isc={ '1', '834'; '2', '834'; '3', '834'; '4', '1250'; '5', '417'; '6', '417'; '7', '417'; '8', '1250'; '9', '417'; '10', '1250'; '11', '417'; '12', '834'; '13', '417'; '14', '417'; '15', '417'; '16', '417'; '17', '1250'; '18', '417'; '19', '834'; '20', '417'; '21', '417'; '23', '834'; '24', '834'; '25', '1250'; '26', '417'; '27', '417'; '28', '417'; '29', '834'; '30', '417' }  Buses_Isc={ '1', '834'; '2', '834'; '3', '834'; '4', '834'; '5', '1250'; '6', '417'; '7', '417'; '8', '417'; '9', '1250'; '10', '1250'; '11', '1250'; '12', '417'; '13', '834'; '14', '417'; '15', '417'; '16', '417'; '17', '834'; '18', '1250'; '19', '417'; '20', '834'; '21', '417'; '22', '417'; '23', '834'; '24', '417'; '25', '834'; '26', '1250'; '27', '417'; '28', '417'; '29', '417'; '30', '834' }
      settings: SourceProductName=ABB UPPAAL Library
  Source_23 : ABB_UPPAAL_Library/Source_1  MyInitialization=0  Source_ID=23  Lines_Isc={ '1', '834'; '2', '834'; '3', '834'; '4', '1250'; '5', '417'; '6', '417'; '7', '417'; '8', '1250'; '9', '417'; '10', '1250'; '11', '417'; '12', '834'; '13', '417'; '14', '417'; '15', '417'; '16', '417'; '17', '1250'; '18', '417'; '19', '834'; '20', '417'; '21', '417'; '23', '834'; '24', '834'; '25', '1250'; '26', '417'; '27', '417'; '28', '417'; '29', '834'; '30', '417' }  Buses_Isc={ '1', '834'; '2', '834'; '3', '834'; '4', '834'; '5', '1250'; '6', '417'; '7', '417'; '8', '417'; '9', '1250'; '10', '1250'; '11', '1250'; '12', '417'; '13', '834'; '14', '417'; '15', '417'; '16', '417'; '17', '834'; '18', '1250'; '19', '417'; '20', '834'; '21', '417'; '22', '417'; '23', '834'; '24', '417'; '25', '834'; '26', '1250'; '27', '417'; '28', '417'; '29', '417'; '30', '834' }
      settings: SourceProductName=ABB UPPAAL Library
  Source_30 : ABB_UPPAAL_Library/Source_1  MyInitialization=0  Source_ID=30  Lines_Isc={ '1', '834'; '2', '834'; '3', '834'; '4', '1250'; '5', '417'; '6', '417'; '7', '417'; '8', '1250'; '9', '417'; '10', '1250'; '11', '417'; '12', '834'; '13', '417'; '14', '417'; '15', '417'; '16', '417'; '17', '1250'; '18', '417'; '19', '834'; '20', '417'; '21', '417'; '23', '834'; '24', '834'; '25', '1250'; '26', '417'; '27', '417'; '28', '417'; '29', '834'; '30', '417' }  Buses_Isc={ '1', '834'; '2', '834'; '3', '834'; '4', '834'; '5', '1250'; '6', '417'; '7', '417'; '8', '417'; '9', '1250'; '10', '1250'; '11', '1250'; '12', '417'; '13', '834'; '14', '417'; '15', '417'; '16', '417'; '17', '834'; '18', '1250'; '19', '417'; '20', '834'; '21', '417'; '22', '417'; '23', '834'; '24', '417'; '25', '834'; '26', '1250'; '27', '417'; '28', '417'; '29', '417'; '30', '834' }
      settings: SourceProductName=ABB UPPAAL Library
  Source_9 : ABB_UPPAAL_Library/Source_1  MyInitialization=0  Source_ID=9  Lines_Isc={ '1', '1250'; '2', '1250'; '3', '1250'; '4', '1875'; '5', '625'; '6', '625'; '7', '625'; '8', '1875'; '9', '625'; '10', '1875'; '11', '625'; '12', '1250'; '13', '625'; '14', '625'; '15', '625'; '16', '625'; '17', '1875'; '18', '625'; '19', '1250'; '20', '625'; '21', '625'; '23', '1250'; '24', '1250'; '25', '1875'; '26', '625'; '27', '625'; '28', '625'; '29', '1250'; '30', '625' }  Buses_Isc={ '1', '1250'; '2', '1250'; '3', '1250'; '4', '1250'; '5', '1875'; '6', '625'; '7', '625'; '8', '625'; '9', '1875'; '10', '1875'; '11', '1875'; '12', '625'; '13', '1250'; '14', '625'; '15', '625'; '16', '625'; '17', '1250'; '18', '1875'; '19', '625'; '20', '1250'; '21', '625'; '22', '625'; '23', '1250'; '24', '625'; '25', '1250'; '26', '1875'; '27', '625'; '28', '625'; '29', '625'; '30', '1250' }
      settings: SourceProductName=ABB UPPAAL Library
  wires:
  CB_12/1 -> Line_12/1
  Bus_5/1(y) -> CB_5/1, CB_7/1, CB_6/1
  CB_7/1 -> Line_7/1
  CB_9/1 -> Bus_10/1(data)
  Bus_12/1(y) -> Load_4/1
  Line_6/1 -> Bus_7/1(u)
  Bus_9/1(y) -> Line_8/1
  Line_12/1 -> Bus_13/1(u)
  Bus_4/1(y) -> Line_9/1, CB_4/1
  CB_14/1 -> Line_14/1
  CB_3/1 -> Bus_4/1(data)
  Line_9/1 -> CB_9/1
  Line_13/1 -> Bus_14/1(u)
  CB_13/1 -> Line_13/1
  CB_5/1 -> Line_5/1
  CB_8/1 -> Bus_10/2(u)
  Source_9/1 -> Bus_9/1(u)
  Bus_6/1(y) -> Load_1/1
  Bus_13/1(y) -> CB_14/1, CB_13/1
  Bus_14/1(y) -> Load_5/1
  CB_10/1 -> Line_10/1
  Bus_11/1(y) -> CB_11/1, CB_12/1
  Line_7/1 -> Bus_8/1(u)
  CB_4/1 -> Line_4/1
  Line_14/1 -> Bus_15/1(u)
  Line_3/1 -> CB_3/1
  CB_1/1 -> Bus_3/1(u)
  Bus_1/1(y) -> Line_1/1
  Bus_8/1(y) -> Load_3/1
  CB_11/1 -> Line_11/1
  Source_2/1 -> Bus_2/1(u)
  Bus_3/1(y) -> Line_3/1
  Line_1/1 -> CB_1/1
  Line_8/1 -> CB_8/1
  Source_1/1 -> Bus_1/1(u)
  Line_4/1 -> Bus_5/1(u)
  Line_11/1 -> Bus_12/1(u)
  Line_2/1 -> CB_2/1
  Bus_15/1(y) -> Load_6/1
  CB_6/1 -> Line_6/1
  CB_2/1 -> Bus_4/2(u)
  Bus_2/1(y) -> Line_2/1
  Line_5/1 -> Bus_6/1(u)
  Bus_7/1(y) -> Load_2/1
  Line_10/1 -> Bus_11/1(u)
  Line_15/1 -> CB_15/1
  CB_15/1 -> Bus_24/1(data)
  Bus_10/1(y) -> Line_15/1, CB_10/1
  CB_26/1 -> Line_27/1
  Line_28/1 -> Bus_29/1(u)
  Line_29/1 -> CB_28/1
  CB_27/1 -> Line_28/1
  CB_17/1 -> Line_17/1
  Bus_19/1(y) -> Load_10/1
  Line_25/1 -> Bus_26/1(u)
  Line_30/1 -> CB_29/1
  CB_25/1 -> Line_26/1
  Bus_25/1(y) -> Line_30/1, CB_24/1
  Line_18/1 -> Bus_19/1(u)
  Bus_27/1(y) -> Load_7/1
  CB_28/1 -> Bus_17/2(u)
  CB_20/1 -> Line_20/1
  Line_19/1 -> Bus_20/1(u)
  Source_23/1 -> Bus_23/1(u)
  CB_18/1 -> Line_18/1
  CB_22/1 -> Bus_25/2(u)
  Bus_30/1(y) -> Line_29/1
  Bus_21/1(y) -> Load_11/1
  Source_16/1 -> Bus_16/1(u)
  Line_16/1 -> CB_16/1
  Bus_29/1(y) -> Load_9/1
  Line_20/1 -> Bus_21/1(u)
  CB_23/1 -> Bus_25/1(data)
  Line_24/1 -> CB_23/1
  Bus_16/1(y) -> Line_16/1
  CB_24/1 -> Line_25/1
  Bus_17/1(y) -> CB_17/1
  Bus_18/1(y) -> CB_18/1, CB_19/1
  CB_29/1 -> Bus_17/1(data)
  Line_17/1 -> Bus_18/1(u)
  Bus_24/1(y) -> Line_24/1
  CB_19/1 -> Line_19/1
  Line_23/1 -> CB_22/1
  Source_30/1 -> Bus_30/1(u)
  CB_16/1 -> Bus_24/2(u)
  Bus_26/1(y) -> CB_25/1, CB_27/1, CB_26/1
  Bus_20/1(y) -> CB_21/1, CB_20/1
  Line_26/1 -> Bus_27/1(u)
  Bus_23/1(y) -> Line_23/1
  Bus_28/1(y) -> Load_8/1
  CB_21/1 -> Line_21/1
  Line_21/1 -> Bus_22/1(u)
  Bus_22/1(y) -> Load_12/1
  Line_27/1 -> Bus_28/1(u)
